simulink model "gm_minutiaeextraction_21821"  (R2018b)
settings: Solver=FixedStepDiscrete  StartTime=0.0  StopTime=10  RelTol=1e-3
undefined symbols (not defined in the file or in its folder): gray
libraries: hdlsllib x4, visionsources x1, dspmtrx3 x1
(part 2 of 7)

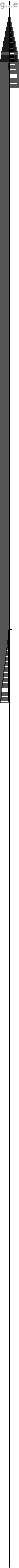
== system gm_minutiaeextraction_21821/MinutiaeFeature ==
  In1 : Inport  OutDataTypeStr=boolean  PortDimensions=[8192]  SampleTime=0.1
  MinutaeExtractTh : Subsystem
  Serializer1D1 : hdlsllib/HDL Operations/Serializer1D  Ratio=1  IdleCycles=0  validIn=off  startOut=off  validOut=off  inputDataDimensions=8192  inputSampleTime=0.1  inputSignalType=real
      settings: SourceProductName=HDL Coder  SourceProductBaseCode=HD
  concatenate{,1..63} (64 alike) : Concatenate  NumInputs=128  ConcatenateDimension=2
  concatenate64 : Concatenate  NumInputs=64  Mode=Multidimensional array  ConcatenateDimension=2
  t : Demux  Outputs=8192
  Out1 : Outport
  wires:
  In1/1 -> Serializer1D1/1
  MinutaeExtractTh/1(Out1) -> Out1/1
  concatenate64/1 -> MinutaeExtractTh/1(In1)
  Serializer1D1/1 -> t/1
  t/1 -> concatenate/1
  t/2 -> concatenate/2
  t/3 -> concatenate/3
  t/4 -> concatenate/4
  t/5 -> concatenate/5
  t/6 -> concatenate/6
  t/7 -> concatenate/7
  t/8 -> concatenate/8
  t/9 -> concatenate/9
  t/10 -> concatenate/10
  t/11 -> concatenate/11
  t/12 -> concatenate/12
  t/13 -> concatenate/13
  t/14 -> concatenate/14
  t/15 -> concatenate/15
  t/16 -> concatenate/16
  t/17 -> concatenate/17
  t/18 -> concatenate/18
  t/19 -> concatenate/19
  t/20 -> concatenate/20
  t/21 -> concatenate/21
  t/22 -> concatenate/22
  t/23 -> concatenate/23
  t/24 -> concatenate/24
  t/25 -> concatenate/25
  t/26 -> concatenate/26
  t/27 -> concatenate/27
  t/28 -> concatenate/28
  t/29 -> concatenate/29
  t/30 -> concatenate/30
  t/31 -> concatenate/31
  t/32 -> concatenate/32
  t/33 -> concatenate/33
  t/34 -> concatenate/34
  t/35 -> concatenate/35
  t/36 -> concatenate/36
  t/37 -> concatenate/37
  t/38 -> concatenate/38
  t/39 -> concatenate/39
  t/40 -> concatenate/40
  t/41 -> concatenate/41
  t/42 -> concatenate/42
  t/43 -> concatenate/43
  t/44 -> concatenate/44
  t/45 -> concatenate/45
  t/46 -> concatenate/46
  t/47 -> concatenate/47
  t/48 -> concatenate/48
  t/49 -> concatenate/49
  t/50 -> concatenate/50
  t/51 -> concatenate/51
  t/52 -> concatenate/52
  t/53 -> concatenate/53
  t/54 -> concatenate/54
  t/55 -> concatenate/55
  t/56 -> concatenate/56
  t/57 -> concatenate/57
  t/58 -> concatenate/58
  t/59 -> concatenate/59
  t/60 -> concatenate/60
  t/61 -> concatenate/61
  t/62 -> concatenate/62
  t/63 -> concatenate/63
  t/64 -> concatenate/64
  t/65 -> concatenate/65
  t/66 -> concatenate/66
  t/67 -> concatenate/67
  t/68 -> concatenate/68
  t/69 -> concatenate/69
  t/70 -> concatenate/70
  t/71 -> concatenate/71
  t/72 -> concatenate/72
  t/73 -> concatenate/73
  t/74 -> concatenate/74
  t/75 -> concatenate/75
  t/76 -> concatenate/76
  t/77 -> concatenate/77
  t/78 -> concatenate/78
  t/79 -> concatenate/79
  t/80 -> concatenate/80
  t/81 -> concatenate/81
  t/82 -> concatenate/82
  t/83 -> concatenate/83
  t/84 -> concatenate/84
  t/85 -> concatenate/85
  t/86 -> concatenate/86
  t/87 -> concatenate/87
  t/88 -> concatenate/88
  t/89 -> concatenate/89
  t/90 -> concatenate/90
  t/91 -> concatenate/91
  t/92 -> concatenate/92
  t/93 -> concatenate/93
  t/94 -> concatenate/94
  t/95 -> concatenate/95
  t/96 -> concatenate/96
  t/97 -> concatenate/97
  t/98 -> concatenate/98
  t/99 -> concatenate/99
  t/100 -> concatenate/100
  t/101 -> concatenate/101
  t/102 -> concatenate/102
  t/103 -> concatenate/103
  t/104 -> concatenate/104
  t/105 -> concatenate/105
  t/106 -> concatenate/106
  t/107 -> concatenate/107
  t/108 -> concatenate/108
  t/109 -> concatenate/109
  t/110 -> concatenate/110
  t/111 -> concatenate/111
  t/112 -> concatenate/112
  t/113 -> concatenate/113
  t/114 -> concatenate/114
  t/115 -> concatenate/115
  t/116 -> concatenate/116
  t/117 -> concatenate/117
  t/118 -> concatenate/118
  t/119 -> concatenate/119
  t/120 -> concatenate/120
  t/121 -> concatenate/121
  t/122 -> concatenate/122
  t/123 -> concatenate/123
  t/124 -> concatenate/124
  t/125 -> concatenate/125
  t/126 -> concatenate/126
  t/127 -> concatenate/127
  t/128 -> concatenate/128
  t/129 -> concatenate1/1
  t/130 -> concatenate1/2
  t/131 -> concatenate1/3
  t/132 -> concatenate1/4
  t/133 -> concatenate1/5
  t/134 -> concatenate1/6
  t/135 -> concatenate1/7
  t/136 -> concatenate1/8
  t/137 -> concatenate1/9
  t/138 -> concatenate1/10
  t/139 -> concatenate1/11
  t/140 -> concatenate1/12
  t/141 -> concatenate1/13
  t/142 -> concatenate1/14
  t/143 -> concatenate1/15
  t/144 -> concatenate1/16
  t/145 -> concatenate1/17
  t/146 -> concatenate1/18
  t/147 -> concatenate1/19
  t/148 -> concatenate1/20
  t/149 -> concatenate1/21
  t/150 -> concatenate1/22
  t/151 -> concatenate1/23
  t/152 -> concatenate1/24
  t/153 -> concatenate1/25
  t/154 -> concatenate1/26
  t/155 -> concatenate1/27
  t/156 -> concatenate1/28
  t/157 -> concatenate1/29
  t/158 -> concatenate1/30
  t/159 -> concatenate1/31
  t/160 -> concatenate1/32
  t/161 -> concatenate1/33
  t/162 -> concatenate1/34
  t/163 -> concatenate1/35
  t/164 -> concatenate1/36
  t/165 -> concatenate1/37
  t/166 -> concatenate1/38
  t/167 -> concatenate1/39
  t/168 -> concatenate1/40
  t/169 -> concatenate1/41
  t/170 -> concatenate1/42
  t/171 -> concatenate1/43
  t/172 -> concatenate1/44
  t/173 -> concatenate1/45
  t/174 -> concatenate1/46
  t/175 -> concatenate1/47
  t/176 -> concatenate1/48
  t/177 -> concatenate1/49
  t/178 -> concatenate1/50
  t/179 -> concatenate1/51
  t/180 -> concatenate1/52
  t/181 -> concatenate1/53
  t/182 -> concatenate1/54
  t/183 -> concatenate1/55
  t/184 -> concatenate1/56
  t/185 -> concatenate1/57
  t/186 -> concatenate1/58
  t/187 -> concatenate1/59
  t/188 -> concatenate1/60
  t/189 -> concatenate1/61
  t/190 -> concatenate1/62
  t/191 -> concatenate1/63
  t/192 -> concatenate1/64
  t/193 -> concatenate1/65
  t/194 -> concatenate1/66
  t/195 -> concatenate1/67
  t/196 -> concatenate1/68
  t/197 -> concatenate1/69
  t/198 -> concatenate1/70
  t/199 -> concatenate1/71
  t/200 -> concatenate1/72
  t/201 -> concatenate1/73
  t/202 -> concatenate1/74
  t/203 -> concatenate1/75
  t/204 -> concatenate1/76
  t/205 -> concatenate1/77
  t/206 -> concatenate1/78
  t/207 -> concatenate1/79
  t/208 -> concatenate1/80
  t/209 -> concatenate1/81
  t/210 -> concatenate1/82
  t/211 -> concatenate1/83
  t/212 -> concatenate1/84
  t/213 -> concatenate1/85
  t/214 -> concatenate1/86
  t/215 -> concatenate1/87
  t/216 -> concatenate1/88
  t/217 -> concatenate1/89
  t/218 -> concatenate1/90
  t/219 -> concatenate1/91
  t/220 -> concatenate1/92
  t/221 -> concatenate1/93
  t/222 -> concatenate1/94
  t/223 -> concatenate1/95
  t/224 -> concatenate1/96
  t/225 -> concatenate1/97
  t/226 -> concatenate1/98
  t/227 -> concatenate1/99
  t/228 -> concatenate1/100
  t/229 -> concatenate1/101
  t/230 -> concatenate1/102
  t/231 -> concatenate1/103
  t/232 -> concatenate1/104
  t/233 -> concatenate1/105
  t/234 -> concatenate1/106
  t/235 -> concatenate1/107
  t/236 -> concatenate1/108
  t/237 -> concatenate1/109
  t/238 -> concatenate1/110
  t/239 -> concatenate1/111
  t/240 -> concatenate1/112
  t/241 -> concatenate1/113
  t/242 -> concatenate1/114
  t/243 -> concatenate1/115
  t/244 -> concatenate1/116
  t/245 -> concatenate1/117
  t/246 -> concatenate1/118
  t/247 -> concatenate1/119
  t/248 -> concatenate1/120
  t/249 -> concatenate1/121
  t/250 -> concatenate1/122
  t/251 -> concatenate1/123
  t/252 -> concatenate1/124
  t/253 -> concatenate1/125
  t/254 -> concatenate1/126
  t/255 -> concatenate1/127
  t/256 -> concatenate1/128
  t/257 -> concatenate2/1
  t/258 -> concatenate2/2
  t/259 -> concatenate2/3
  t/260 -> concatenate2/4
  t/261 -> concatenate2/5
  t/262 -> concatenate2/6
  t/263 -> concatenate2/7
  t/264 -> concatenate2/8
  t/265 -> concatenate2/9
  t/266 -> concatenate2/10
  t/267 -> concatenate2/11
  t/268 -> concatenate2/12
  t/269 -> concatenate2/13
  t/270 -> concatenate2/14
  t/271 -> concatenate2/15
  t/272 -> concatenate2/16
  t/273 -> concatenate2/17
  t/274 -> concatenate2/18
  t/275 -> concatenate2/19
  t/276 -> concatenate2/20
  t/277 -> concatenate2/21
  t/278 -> concatenate2/22
  t/279 -> concatenate2/23
  t/280 -> concatenate2/24
  t/281 -> concatenate2/25
  t/282 -> concatenate2/26
  t/283 -> concatenate2/27
  t/284 -> concatenate2/28
  t/285 -> concatenate2/29
  t/286 -> concatenate2/30
  t/287 -> concatenate2/31
  t/288 -> concatenate2/32
  t/289 -> concatenate2/33
  t/290 -> concatenate2/34
  t/291 -> concatenate2/35
  t/292 -> concatenate2/36
  t/293 -> concatenate2/37
  t/294 -> concatenate2/38
  t/295 -> concatenate2/39
  t/296 -> concatenate2/40
  t/297 -> concatenate2/41
  t/298 -> concatenate2/42
  t/299 -> concatenate2/43
  t/300 -> concatenate2/44
  t/301 -> concatenate2/45
  t/302 -> concatenate2/46
  t/303 -> concatenate2/47
  t/304 -> concatenate2/48
  t/305 -> concatenate2/49
  t/306 -> concatenate2/50
  t/307 -> concatenate2/51
  t/308 -> concatenate2/52
  t/309 -> concatenate2/53
  t/310 -> concatenate2/54
  t/311 -> concatenate2/55
  t/312 -> concatenate2/56
  t/313 -> concatenate2/57
  t/314 -> concatenate2/58
  t/315 -> concatenate2/59
  t/316 -> concatenate2/60
  t/317 -> concatenate2/61
  t/318 -> concatenate2/62
  t/319 -> concatenate2/63
  t/320 -> concatenate2/64
  t/321 -> concatenate2/65
  t/322 -> concatenate2/66
  t/323 -> concatenate2/67
  t/324 -> concatenate2/68
  t/325 -> concatenate2/69
  t/326 -> concatenate2/70
  t/327 -> concatenate2/71
  t/328 -> concatenate2/72
  t/329 -> concatenate2/73
  t/330 -> concatenate2/74
  t/331 -> concatenate2/75
  t/332 -> concatenate2/76
  t/333 -> concatenate2/77
  t/334 -> concatenate2/78
  t/335 -> concatenate2/79
  t/336 -> concatenate2/80
  t/337 -> concatenate2/81
  t/338 -> concatenate2/82
  t/339 -> concatenate2/83
  t/340 -> concatenate2/84
  t/341 -> concatenate2/85
  t/342 -> concatenate2/86
  t/343 -> concatenate2/87
  t/344 -> concatenate2/88
  t/345 -> concatenate2/89
  t/346 -> concatenate2/90
  t/347 -> concatenate2/91
  t/348 -> concatenate2/92
  t/349 -> concatenate2/93
  t/350 -> concatenate2/94
  t/351 -> concatenate2/95
  t/352 -> concatenate2/96
  t/353 -> concatenate2/97
  t/354 -> concatenate2/98
  t/355 -> concatenate2/99
  t/356 -> concatenate2/100
  t/357 -> concatenate2/101
  t/358 -> concatenate2/102
  t/359 -> concatenate2/103
  t/360 -> concatenate2/104
  t/361 -> concatenate2/105
  t/362 -> concatenate2/106
  t/363 -> concatenate2/107
  t/364 -> concatenate2/108
  t/365 -> concatenate2/109
  t/366 -> concatenate2/110
  t/367 -> concatenate2/111
  t/368 -> concatenate2/112
  t/369 -> concatenate2/113
  t/370 -> concatenate2/114
  t/371 -> concatenate2/115
  t/372 -> concatenate2/116
  t/373 -> concatenate2/117
  t/374 -> concatenate2/118
  t/375 -> concatenate2/119
  t/376 -> concatenate2/120
  t/377 -> concatenate2/121
  t/378 -> concatenate2/122
  t/379 -> concatenate2/123
  t/380 -> concatenate2/124
  t/381 -> concatenate2/125
  t/382 -> concatenate2/126
  t/383 -> concatenate2/127
  t/384 -> concatenate2/128
  t/385 -> concatenate3/1
  t/386 -> concatenate3/2
  t/387 -> concatenate3/3
  t/388 -> concatenate3/4
  t/389 -> concatenate3/5
  t/390 -> concatenate3/6
  t/391 -> concatenate3/7
  t/392 -> concatenate3/8
  t/393 -> concatenate3/9
  t/394 -> concatenate3/10
  t/395 -> concatenate3/11
  t/396 -> concatenate3/12
  t/397 -> concatenate3/13
  t/398 -> concatenate3/14
  t/399 -> concatenate3/15
  t/400 -> concatenate3/16
  t/401 -> concatenate3/17
  t/402 -> concatenate3/18
  t/403 -> concatenate3/19
  t/404 -> concatenate3/20
  t/405 -> concatenate3/21
  t/406 -> concatenate3/22
  t/407 -> concatenate3/23
  t/408 -> concatenate3/24
  t/409 -> concatenate3/25
  t/410 -> concatenate3/26
  t/411 -> concatenate3/27
  t/412 -> concatenate3/28
  t/413 -> concatenate3/29
  t/414 -> concatenate3/30
  t/415 -> concatenate3/31
  t/416 -> concatenate3/32
  t/417 -> concatenate3/33
  t/418 -> concatenate3/34
  t/419 -> concatenate3/35
  t/420 -> concatenate3/36
  t/421 -> concatenate3/37
  t/422 -> concatenate3/38
  t/423 -> concatenate3/39
  t/424 -> concatenate3/40
  t/425 -> concatenate3/41
  t/426 -> concatenate3/42
  t/427 -> concatenate3/43
  t/428 -> concatenate3/44
  t/429 -> concatenate3/45
  t/430 -> concatenate3/46
  t/431 -> concatenate3/47
  t/432 -> concatenate3/48
  t/433 -> concatenate3/49
  t/434 -> concatenate3/50
  t/435 -> concatenate3/51
  t/436 -> concatenate3/52
  t/437 -> concatenate3/53
  t/438 -> concatenate3/54
  t/439 -> concatenate3/55
  t/440 -> concatenate3/56
  t/441 -> concatenate3/57
  t/442 -> concatenate3/58
  t/443 -> concatenate3/59
  t/444 -> concatenate3/60
  t/445 -> concatenate3/61
  t/446 -> concatenate3/62
  t/447 -> concatenate3/63
  t/448 -> concatenate3/64
  t/449 -> concatenate3/65
  t/450 -> concatenate3/66
  t/451 -> concatenate3/67
  t/452 -> concatenate3/68
  t/453 -> concatenate3/69
  t/454 -> concatenate3/70
  t/455 -> concatenate3/71
  t/456 -> concatenate3/72
  t/457 -> concatenate3/73
  t/458 -> concatenate3/74
  t/459 -> concatenate3/75
  t/460 -> concatenate3/76
  t/461 -> concatenate3/77
  t/462 -> concatenate3/78
  t/463 -> concatenate3/79
  t/464 -> concatenate3/80
  t/465 -> concatenate3/81
  t/466 -> concatenate3/82
  t/467 -> concatenate3/83
  t/468 -> concatenate3/84
  t/469 -> concatenate3/85
  t/470 -> concatenate3/86
  t/471 -> concatenate3/87
  t/472 -> concatenate3/88
  t/473 -> concatenate3/89
  t/474 -> concatenate3/90
  t/475 -> concatenate3/91
  t/476 -> concatenate3/92
  t/477 -> concatenate3/93
  t/478 -> concatenate3/94
  t/479 -> concatenate3/95
  t/480 -> concatenate3/96
  t/481 -> concatenate3/97
  t/482 -> concatenate3/98
  t/483 -> concatenate3/99
  t/484 -> concatenate3/100
  t/485 -> concatenate3/101
  t/486 -> concatenate3/102
  t/487 -> concatenate3/103
  t/488 -> concatenate3/104
  t/489 -> concatenate3/105
  t/490 -> concatenate3/106
  t/491 -> concatenate3/107
  t/492 -> concatenate3/108
  t/493 -> concatenate3/109
  t/494 -> concatenate3/110
  t/495 -> concatenate3/111
  t/496 -> concatenate3/112
  t/497 -> concatenate3/113
  t/498 -> concatenate3/114
  t/499 -> concatenate3/115
  t/500 -> concatenate3/116
  t/501 -> concatenate3/117
  t/502 -> concatenate3/118
  t/503 -> concatenate3/119
  t/504 -> concatenate3/120
  t/505 -> concatenate3/121
  t/506 -> concatenate3/122
  t/507 -> concatenate3/123
  t/508 -> concatenate3/124
  t/509 -> concatenate3/125
  t/510 -> concatenate3/126
  t/511 -> concatenate3/127
  t/512 -> concatenate3/128
  t/513 -> concatenate4/1
  t/514 -> concatenate4/2
  t/515 -> concatenate4/3
  t/516 -> concatenate4/4
  t/517 -> concatenate4/5
  t/518 -> concatenate4/6
  t/519 -> concatenate4/7
  t/520 -> concatenate4/8
  t/521 -> concatenate4/9
  t/522 -> concatenate4/10
  t/523 -> concatenate4/11
  t/524 -> concatenate4/12
  t/525 -> concatenate4/13
  t/526 -> concatenate4/14
  t/527 -> concatenate4/15
  t/528 -> concatenate4/16
  t/529 -> concatenate4/17
  t/530 -> concatenate4/18
  t/531 -> concatenate4/19
  t/532 -> concatenate4/20
  t/533 -> concatenate4/21
  t/534 -> concatenate4/22
  t/535 -> concatenate4/23
  t/536 -> concatenate4/24
  t/537 -> concatenate4/25
  t/538 -> concatenate4/26
  t/539 -> concatenate4/27
  t/540 -> concatenate4/28
  t/541 -> concatenate4/29
  t/542 -> concatenate4/30
  t/543 -> concatenate4/31
  t/544 -> concatenate4/32
  t/545 -> concatenate4/33
  t/546 -> concatenate4/34
  t/547 -> concatenate4/35
  t/548 -> concatenate4/36
  t/549 -> concatenate4/37
  t/550 -> concatenate4/38
  t/551 -> concatenate4/39
  t/552 -> concatenate4/40
  t/553 -> concatenate4/41
  t/554 -> concatenate4/42
  t/555 -> concatenate4/43
  t/556 -> concatenate4/44
  t/557 -> concatenate4/45
  t/558 -> concatenate4/46
  t/559 -> concatenate4/47
  t/560 -> concatenate4/48
  t/561 -> concatenate4/49
  t/562 -> concatenate4/50
  t/563 -> concatenate4/51
  t/564 -> concatenate4/52
  t/565 -> concatenate4/53
  t/566 -> concatenate4/54
  t/567 -> concatenate4/55
  t/568 -> concatenate4/56
  t/569 -> concatenate4/57
  t/570 -> concatenate4/58
  t/571 -> concatenate4/59
  t/572 -> concatenate4/60
  t/573 -> concatenate4/61
  t/574 -> concatenate4/62
  t/575 -> concatenate4/63
  t/576 -> concatenate4/64
  t/577 -> concatenate4/65
  t/578 -> concatenate4/66
  t/579 -> concatenate4/67
  t/580 -> concatenate4/68
  t/581 -> concatenate4/69
  t/582 -> concatenate4/70
  t/583 -> concatenate4/71
  t/584 -> concatenate4/72
  t/585 -> concatenate4/73
  t/586 -> concatenate4/74
  t/587 -> concatenate4/75
  t/588 -> concatenate4/76
  t/589 -> concatenate4/77
  t/590 -> concatenate4/78
  t/591 -> concatenate4/79
  t/592 -> concatenate4/80
  t/593 -> concatenate4/81
  t/594 -> concatenate4/82
  t/595 -> concatenate4/83
  t/596 -> concatenate4/84
  t/597 -> concatenate4/85
  t/598 -> concatenate4/86
  t/599 -> concatenate4/87
  t/600 -> concatenate4/88
  t/601 -> concatenate4/89
  t/602 -> concatenate4/90
  t/603 -> concatenate4/91
  t/604 -> concatenate4/92
  t/605 -> concatenate4/93
  t/606 -> concatenate4/94
  t/607 -> concatenate4/95
  t/608 -> concatenate4/96
  t/609 -> concatenate4/97
  t/610 -> concatenate4/98
  t/611 -> concatenate4/99
  t/612 -> concatenate4/100
  t/613 -> concatenate4/101
  t/614 -> concatenate4/102
  t/615 -> concatenate4/103
  t/616 -> concatenate4/104
  t/617 -> concatenate4/105
  t/618 -> concatenate4/106
  t/619 -> concatenate4/107
  t/620 -> concatenate4/108
  t/621 -> concatenate4/109
  t/622 -> concatenate4/110
  t/623 -> concatenate4/111
  t/624 -> concatenate4/112
  t/625 -> concatenate4/113
  t/626 -> concatenate4/114
  t/627 -> concatenate4/115
  t/628 -> concatenate4/116
  t/629 -> concatenate4/117
  t/630 -> concatenate4/118
  t/631 -> concatenate4/119
  t/632 -> concatenate4/120
  t/633 -> concatenate4/121
  t/634 -> concatenate4/122
  t/635 -> concatenate4/123
  t/636 -> concatenate4/124
  t/637 -> concatenate4/125
  t/638 -> concatenate4/126
  t/639 -> concatenate4/127
  t/640 -> concatenate4/128
  t/641 -> concatenate5/1
  t/642 -> concatenate5/2
  t/643 -> concatenate5/3
  t/644 -> concatenate5/4
  t/645 -> concatenate5/5
  t/646 -> concatenate5/6
  t/647 -> concatenate5/7
  t/648 -> concatenate5/8
  t/649 -> concatenate5/9
  t/650 -> concatenate5/10
  t/651 -> concatenate5/11
  t/652 -> concatenate5/12
  t/653 -> concatenate5/13
  t/654 -> concatenate5/14
  t/655 -> concatenate5/15
  t/656 -> concatenate5/16
  t/657 -> concatenate5/17
  t/658 -> concatenate5/18
  t/659 -> concatenate5/19
  t/660 -> concatenate5/20
  t/661 -> concatenate5/21
  t/662 -> concatenate5/22
  t/663 -> concatenate5/23
  t/664 -> concatenate5/24
  t/665 -> concatenate5/25
  t/666 -> concatenate5/26
  t/667 -> concatenate5/27
  t/668 -> concatenate5/28
  t/669 -> concatenate5/29
  t/670 -> concatenate5/30
  t/671 -> concatenate5/31
  t/672 -> concatenate5/32
  t/673 -> concatenate5/33
  t/674 -> concatenate5/34
  t/675 -> concatenate5/35
  t/676 -> concatenate5/36
  t/677 -> concatenate5/37
  t/678 -> concatenate5/38
  t/679 -> concatenate5/39
  t/680 -> concatenate5/40
  t/681 -> concatenate5/41
  t/682 -> concatenate5/42
  t/683 -> concatenate5/43
  t/684 -> concatenate5/44
  t/685 -> concatenate5/45
  t/686 -> concatenate5/46
  t/687 -> concatenate5/47
  t/688 -> concatenate5/48
  t/689 -> concatenate5/49
  t/690 -> concatenate5/50
  t/691 -> concatenate5/51
  t/692 -> concatenate5/52
  t/693 -> concatenate5/53
  t/694 -> concatenate5/54
  t/695 -> concatenate5/55
  t/696 -> concatenate5/56
  t/697 -> concatenate5/57
  t/698 -> concatenate5/58
  t/699 -> concatenate5/59
  t/700 -> concatenate5/60
  t/701 -> concatenate5/61
  t/702 -> concatenate5/62
  t/703 -> concatenate5/63
  t/704 -> concatenate5/64
  t/705 -> concatenate5/65
  t/706 -> concatenate5/66
  t/707 -> concatenate5/67
  t/708 -> concatenate5/68
  t/709 -> concatenate5/69
  t/710 -> concatenate5/70
  t/711 -> concatenate5/71
  t/712 -> concatenate5/72
  t/713 -> concatenate5/73
  t/714 -> concatenate5/74
  t/715 -> concatenate5/75
  t/716 -> concatenate5/76
  t/717 -> concatenate5/77
  t/718 -> concatenate5/78
  t/719 -> concatenate5/79
  t/720 -> concatenate5/80
  t/721 -> concatenate5/81
  t/722 -> concatenate5/82
  t/723 -> concatenate5/83
  t/724 -> concatenate5/84
  t/725 -> concatenate5/85
  t/726 -> concatenate5/86
  t/727 -> concatenate5/87
  t/728 -> concatenate5/88
  t/729 -> concatenate5/89
  t/730 -> concatenate5/90
  t/731 -> concatenate5/91
  t/732 -> concatenate5/92
  t/733 -> concatenate5/93
  t/734 -> concatenate5/94
  t/735 -> concatenate5/95
  t/736 -> concatenate5/96
  t/737 -> concatenate5/97
  t/738 -> concatenate5/98
  t/739 -> concatenate5/99
  t/740 -> concatenate5/100
  t/741 -> concatenate5/101
  t/742 -> concatenate5/102
  t/743 -> concatenate5/103
  t/744 -> concatenate5/104
  t/745 -> concatenate5/105
  t/746 -> concatenate5/106
  t/747 -> concatenate5/107
  t/748 -> concatenate5/108
  t/749 -> concatenate5/109
  t/750 -> concatenate5/110
  t/751 -> concatenate5/111
  t/752 -> concatenate5/112
  t/753 -> concatenate5/113
  t/754 -> concatenate5/114
  t/755 -> concatenate5/115
  t/756 -> concatenate5/116
  t/757 -> concatenate5/117
  t/758 -> concatenate5/118
  t/759 -> concatenate5/119
  t/760 -> concatenate5/120
  t/761 -> concatenate5/121
  t/762 -> concatenate5/122
  t/763 -> concatenate5/123
  t/764 -> concatenate5/124
  t/765 -> concatenate5/125
  t/766 -> concatenate5/126
  t/767 -> concatenate5/127
  t/768 -> concatenate5/128
  t/769 -> concatenate6/1
  t/770 -> concatenate6/2
  t/771 -> concatenate6/3
  t/772 -> concatenate6/4
  t/773 -> concatenate6/5
  t/774 -> concatenate6/6
  t/775 -> concatenate6/7
  t/776 -> concatenate6/8
  t/777 -> concatenate6/9
  t/778 -> concatenate6/10
  t/779 -> concatenate6/11
  t/780 -> concatenate6/12
  t/781 -> concatenate6/13
  t/782 -> concatenate6/14
  t/783 -> concatenate6/15
  t/784 -> concatenate6/16
  t/785 -> concatenate6/17
  t/786 -> concatenate6/18
  t/787 -> concatenate6/19
  t/788 -> concatenate6/20
  t/789 -> concatenate6/21
  t/790 -> concatenate6/22
  t/791 -> concatenate6/23
  t/792 -> concatenate6/24
  t/793 -> concatenate6/25
  t/794 -> concatenate6/26
  t/795 -> concatenate6/27
  t/796 -> concatenate6/28
  t/797 -> concatenate6/29
  t/798 -> concatenate6/30
  t/799 -> concatenate6/31
  t/800 -> concatenate6/32
  t/801 -> concatenate6/33
  t/802 -> concatenate6/34
  t/803 -> concatenate6/35
  t/804 -> concatenate6/36
  t/805 -> concatenate6/37
  t/806 -> concatenate6/38
  t/807 -> concatenate6/39
  t/808 -> concatenate6/40
  t/809 -> concatenate6/41
  t/810 -> concatenate6/42
  t/811 -> concatenate6/43
  t/812 -> concatenate6/44
  t/813 -> concatenate6/45
  t/814 -> concatenate6/46
  t/815 -> concatenate6/47
  t/816 -> concatenate6/48
  t/817 -> concatenate6/49
  t/818 -> concatenate6/50
  t/819 -> concatenate6/51
  t/820 -> concatenate6/52
  t/821 -> concatenate6/53
  t/822 -> concatenate6/54
  t/823 -> concatenate6/55
  t/824 -> concatenate6/56
  t/825 -> concatenate6/57
  t/826 -> concatenate6/58
  t/827 -> concatenate6/59
  t/828 -> concatenate6/60
  t/829 -> concatenate6/61
  t/830 -> concatenate6/62
  t/831 -> concatenate6/63
  t/832 -> concatenate6/64
  t/833 -> concatenate6/65
  t/834 -> concatenate6/66
  t/835 -> concatenate6/67
  t/836 -> concatenate6/68
  t/837 -> concatenate6/69
  t/838 -> concatenate6/70
  t/839 -> concatenate6/71
  t/840 -> concatenate6/72
  t/841 -> concatenate6/73
  t/842 -> concatenate6/74
  t/843 -> concatenate6/75
  t/844 -> concatenate6/76
  t/845 -> concatenate6/77
  t/846 -> concatenate6/78
  t/847 -> concatenate6/79
  t/848 -> concatenate6/80
  t/849 -> concatenate6/81
  t/850 -> concatenate6/82
  t/851 -> concatenate6/83
  t/852 -> concatenate6/84
  t/853 -> concatenate6/85
  t/854 -> concatenate6/86
  t/855 -> concatenate6/87
  t/856 -> concatenate6/88
  t/857 -> concatenate6/89
  t/858 -> concatenate6/90
  t/859 -> concatenate6/91
  t/860 -> concatenate6/92
  t/861 -> concatenate6/93
  t/862 -> concatenate6/94
  t/863 -> concatenate6/95
  t/864 -> concatenate6/96
  t/865 -> concatenate6/97
  t/866 -> concatenate6/98
  t/867 -> concatenate6/99
  t/868 -> concatenate6/100
  t/869 -> concatenate6/101
  t/870 -> concatenate6/102
  t/871 -> concatenate6/103
  t/872 -> concatenate6/104
  t/873 -> concatenate6/105
  t/874 -> concatenate6/106
  t/875 -> concatenate6/107
  t/876 -> concatenate6/108
  t/877 -> concatenate6/109
  t/878 -> concatenate6/110
  t/879 -> concatenate6/111
  t/880 -> concatenate6/112
  t/881 -> concatenate6/113
  t/882 -> concatenate6/114
  t/883 -> concatenate6/115
  t/884 -> concatenate6/116
  t/885 -> concatenate6/117
  t/886 -> concatenate6/118
  t/887 -> concatenate6/119
  t/888 -> concatenate6/120
  t/889 -> concatenate6/121
  t/890 -> concatenate6/122
  t/891 -> concatenate6/123
  t/892 -> concatenate6/124
  t/893 -> concatenate6/125
  t/894 -> concatenate6/126
  t/895 -> concatenate6/127
  t/896 -> concatenate6/128
  t/897 -> concatenate7/1
  t/898 -> concatenate7/2
  t/899 -> concatenate7/3
  t/900 -> concatenate7/4
  t/901 -> concatenate7/5
  t/902 -> concatenate7/6
  t/903 -> concatenate7/7
  t/904 -> concatenate7/8
  t/905 -> concatenate7/9
  t/906 -> concatenate7/10
  t/907 -> concatenate7/11
  t/908 -> concatenate7/12
  t/909 -> concatenate7/13
  t/910 -> concatenate7/14
  t/911 -> concatenate7/15
  t/912 -> concatenate7/16
  t/913 -> concatenate7/17
  t/914 -> concatenate7/18
  t/915 -> concatenate7/19
  t/916 -> concatenate7/20
  t/917 -> concatenate7/21
  t/918 -> concatenate7/22
  t/919 -> concatenate7/23
  t/920 -> concatenate7/24
  t/921 -> concatenate7/25
  t/922 -> concatenate7/26
  t/923 -> concatenate7/27
  t/924 -> concatenate7/28
  t/925 -> concatenate7/29
  t/926 -> concatenate7/30
  t/927 -> concatenate7/31
  t/928 -> concatenate7/32
  t/929 -> concatenate7/33
  t/930 -> concatenate7/34
  t/931 -> concatenate7/35
  t/932 -> concatenate7/36
  t/933 -> concatenate7/37
  t/934 -> concatenate7/38
  t/935 -> concatenate7/39
  t/936 -> concatenate7/40
  t/937 -> concatenate7/41
  t/938 -> concatenate7/42
  t/939 -> concatenate7/43
  t/940 -> concatenate7/44
  t/941 -> concatenate7/45
  t/942 -> concatenate7/46
  t/943 -> concatenate7/47
  t/944 -> concatenate7/48
  t/945 -> concatenate7/49
  t/946 -> concatenate7/50
  t/947 -> concatenate7/51
  t/948 -> concatenate7/52
  t/949 -> concatenate7/53
  t/950 -> concatenate7/54
  t/951 -> concatenate7/55
  t/952 -> concatenate7/56
  t/953 -> concatenate7/57
  t/954 -> concatenate7/58
  t/955 -> concatenate7/59
  t/956 -> concatenate7/60
  t/957 -> concatenate7/61
  t/958 -> concatenate7/62
  t/959 -> concatenate7/63
  t/960 -> concatenate7/64
  t/961 -> concatenate7/65
  t/962 -> concatenate7/66
  t/963 -> concatenate7/67
  t/964 -> concatenate7/68
  t/965 -> concatenate7/69
  t/966 -> concatenate7/70
  t/967 -> concatenate7/71
  t/968 -> concatenate7/72
  t/969 -> concatenate7/73
  t/970 -> concatenate7/74
  t/971 -> concatenate7/75
  t/972 -> concatenate7/76
  t/973 -> concatenate7/77
  t/974 -> concatenate7/78
  t/975 -> concatenate7/79
  t/976 -> concatenate7/80
  t/977 -> concatenate7/81
  t/978 -> concatenate7/82
  t/979 -> concatenate7/83
  t/980 -> concatenate7/84
  t/981 -> concatenate7/85
  t/982 -> concatenate7/86
  t/983 -> concatenate7/87
  t/984 -> concatenate7/88
  t/985 -> concatenate7/89
  t/986 -> concatenate7/90
  t/987 -> concatenate7/91
  t/988 -> concatenate7/92
  t/989 -> concatenate7/93
  t/990 -> concatenate7/94
  t/991 -> concatenate7/95
  t/992 -> concatenate7/96
  t/993 -> concatenate7/97
  t/994 -> concatenate7/98
  t/995 -> concatenate7/99
  t/996 -> concatenate7/100
  t/997 -> concatenate7/101
  t/998 -> concatenate7/102
  t/999 -> concatenate7/103
  t/1000 -> concatenate7/104
  t/1001 -> concatenate7/105
  t/1002 -> concatenate7/106
  t/1003 -> concatenate7/107
  t/1004 -> concatenate7/108
  t/1005 -> concatenate7/109
  t/1006 -> concatenate7/110
  t/1007 -> concatenate7/111
  t/1008 -> concatenate7/112
  t/1009 -> concatenate7/113
  t/1010 -> concatenate7/114
  t/1011 -> concatenate7/115
  t/1012 -> concatenate7/116
  t/1013 -> concatenate7/117
  t/1014 -> concatenate7/118
  t/1015 -> concatenate7/119
  t/1016 -> concatenate7/120
  t/1017 -> concatenate7/121
  t/1018 -> concatenate7/122
  t/1019 -> concatenate7/123
  t/1020 -> concatenate7/124
  t/1021 -> concatenate7/125
  t/1022 -> concatenate7/126
  t/1023 -> concatenate7/127
  t/1024 -> concatenate7/128
  t/1025 -> concatenate8/1
  t/1026 -> concatenate8/2
  t/1027 -> concatenate8/3
  t/1028 -> concatenate8/4
  t/1029 -> concatenate8/5
  t/1030 -> concatenate8/6
  t/1031 -> concatenate8/7
  t/1032 -> concatenate8/8
  t/1033 -> concatenate8/9
  t/1034 -> concatenate8/10
  t/1035 -> concatenate8/11
  t/1036 -> concatenate8/12
  t/1037 -> concatenate8/13
  t/1038 -> concatenate8/14
  t/1039 -> concatenate8/15
  t/1040 -> concatenate8/16
  t/1041 -> concatenate8/17
  t/1042 -> concatenate8/18
  t/1043 -> concatenate8/19
  t/1044 -> concatenate8/20
  t/1045 -> concatenate8/21
  t/1046 -> concatenate8/22
  t/1047 -> concatenate8/23
  t/1048 -> concatenate8/24
  t/1049 -> concatenate8/25
  t/1050 -> concatenate8/26
  t/1051 -> concatenate8/27
  t/1052 -> concatenate8/28
  t/1053 -> concatenate8/29
  t/1054 -> concatenate8/30
  t/1055 -> concatenate8/31
  t/1056 -> concatenate8/32
  t/1057 -> concatenate8/33
  t/1058 -> concatenate8/34
  t/1059 -> concatenate8/35
  t/1060 -> concatenate8/36
  t/1061 -> concatenate8/37
  t/1062 -> concatenate8/38
  t/1063 -> concatenate8/39
  t/1064 -> concatenate8/40
  t/1065 -> concatenate8/41
  t/1066 -> concatenate8/42
  t/1067 -> concatenate8/43
  t/1068 -> concatenate8/44
  t/1069 -> concatenate8/45
  t/1070 -> concatenate8/46
  t/1071 -> concatenate8/47
  t/1072 -> concatenate8/48
  t/1073 -> concatenate8/49
  t/1074 -> concatenate8/50
  t/1075 -> concatenate8/51
  t/1076 -> concatenate8/52
  t/1077 -> concatenate8/53
  t/1078 -> concatenate8/54
  t/1079 -> concatenate8/55
  t/1080 -> concatenate8/56
  t/1081 -> concatenate8/57
  t/1082 -> concatenate8/58
  t/1083 -> concatenate8/59
  t/1084 -> concatenate8/60
  t/1085 -> concatenate8/61
  t/1086 -> concatenate8/62
  t/1087 -> concatenate8/63
  t/1088 -> concatenate8/64
  t/1089 -> concatenate8/65
  t/1090 -> concatenate8/66
  t/1091 -> concatenate8/67
  t/1092 -> concatenate8/68
  t/1093 -> concatenate8/69
  t/1094 -> concatenate8/70
  t/1095 -> concatenate8/71
  t/1096 -> concatenate8/72
  t/1097 -> concatenate8/73
  t/1098 -> concatenate8/74
  t/1099 -> concatenate8/75
  t/1100 -> concatenate8/76
  t/1101 -> concatenate8/77
  t/1102 -> concatenate8/78
  t/1103 -> concatenate8/79
  t/1104 -> concatenate8/80
  t/1105 -> concatenate8/81
  t/1106 -> concatenate8/82
  t/1107 -> concatenate8/83
  t/1108 -> concatenate8/84
  t/1109 -> concatenate8/85
  t/1110 -> concatenate8/86
  t/1111 -> concatenate8/87
  t/1112 -> concatenate8/88
  t/1113 -> concatenate8/89
  t/1114 -> concatenate8/90
  t/1115 -> concatenate8/91
  t/1116 -> concatenate8/92
  t/1117 -> concatenate8/93
  t/1118 -> concatenate8/94
  t/1119 -> concatenate8/95
  t/1120 -> concatenate8/96
  t/1121 -> concatenate8/97
  t/1122 -> concatenate8/98
  t/1123 -> concatenate8/99
  t/1124 -> concatenate8/100
  t/1125 -> concatenate8/101
  t/1126 -> concatenate8/102
  t/1127 -> concatenate8/103
  t/1128 -> concatenate8/104
  t/1129 -> concatenate8/105
  t/1130 -> concatenate8/106
  t/1131 -> concatenate8/107
  t/1132 -> concatenate8/108
  t/1133 -> concatenate8/109
  t/1134 -> concatenate8/110
  t/1135 -> concatenate8/111
  t/1136 -> concatenate8/112
  t/1137 -> concatenate8/113
  t/1138 -> concatenate8/114
  t/1139 -> concatenate8/115
  t/1140 -> concatenate8/116
  t/1141 -> concatenate8/117
  t/1142 -> concatenate8/118
  t/1143 -> concatenate8/119
  t/1144 -> concatenate8/120
  t/1145 -> concatenate8/121
  t/1146 -> concatenate8/122
  t/1147 -> concatenate8/123
  t/1148 -> concatenate8/124
  t/1149 -> concatenate8/125
  t/1150 -> concatenate8/126
  t/1151 -> concatenate8/127
  t/1152 -> concatenate8/128
  t/1153 -> concatenate9/1
  t/1154 -> concatenate9/2
  t/1155 -> concatenate9/3
  t/1156 -> concatenate9/4
  t/1157 -> concatenate9/5
  t/1158 -> concatenate9/6
  t/1159 -> concatenate9/7
  t/1160 -> concatenate9/8
  t/1161 -> concatenate9/9
  t/1162 -> concatenate9/10
  t/1163 -> concatenate9/11
  t/1164 -> concatenate9/12
  t/1165 -> concatenate9/13
  t/1166 -> concatenate9/14
  t/1167 -> concatenate9/15
  t/1168 -> concatenate9/16
  t/1169 -> concatenate9/17
  t/1170 -> concatenate9/18
  t/1171 -> concatenate9/19
  t/1172 -> concatenate9/20
  t/1173 -> concatenate9/21
  t/1174 -> concatenate9/22
  t/1175 -> concatenate9/23
  t/1176 -> concatenate9/24
  t/1177 -> concatenate9/25
  t/1178 -> concatenate9/26
  t/1179 -> concatenate9/27
  t/1180 -> concatenate9/28
  t/1181 -> concatenate9/29
  t/1182 -> concatenate9/30
  t/1183 -> concatenate9/31
  t/1184 -> concatenate9/32
  t/1185 -> concatenate9/33
  t/1186 -> concatenate9/34
  t/1187 -> concatenate9/35
  t/1188 -> concatenate9/36
  t/1189 -> concatenate9/37
  t/1190 -> concatenate9/38
  t/1191 -> concatenate9/39
  t/1192 -> concatenate9/40
  t/1193 -> concatenate9/41
  t/1194 -> concatenate9/42
  t/1195 -> concatenate9/43
  t/1196 -> concatenate9/44
  t/1197 -> concatenate9/45
  t/1198 -> concatenate9/46
  t/1199 -> concatenate9/47
  t/1200 -> concatenate9/48
  t/1201 -> concatenate9/49
  t/1202 -> concatenate9/50
  t/1203 -> concatenate9/51
  t/1204 -> concatenate9/52
  t/1205 -> concatenate9/53
  t/1206 -> concatenate9/54
  t/1207 -> concatenate9/55
  t/1208 -> concatenate9/56
  t/1209 -> concatenate9/57
  t/1210 -> concatenate9/58
  t/1211 -> concatenate9/59
  t/1212 -> concatenate9/60
  t/1213 -> concatenate9/61
  t/1214 -> concatenate9/62
  t/1215 -> concatenate9/63
  t/1216 -> concatenate9/64
  t/1217 -> concatenate9/65
  t/1218 -> concatenate9/66
  t/1219 -> concatenate9/67
  t/1220 -> concatenate9/68
  t/1221 -> concatenate9/69
  t/1222 -> concatenate9/70
  t/1223 -> concatenate9/71
  t/1224 -> concatenate9/72
  t/1225 -> concatenate9/73
  t/1226 -> concatenate9/74
  t/1227 -> concatenate9/75
  t/1228 -> concatenate9/76
  t/1229 -> concatenate9/77
  t/1230 -> concatenate9/78
  t/1231 -> concatenate9/79
  t/1232 -> concatenate9/80
  t/1233 -> concatenate9/81
  t/1234 -> concatenate9/82
  t/1235 -> concatenate9/83
  t/1236 -> concatenate9/84
  t/1237 -> concatenate9/85
  t/1238 -> concatenate9/86
  t/1239 -> concatenate9/87
  t/1240 -> concatenate9/88
  t/1241 -> concatenate9/89
  t/1242 -> concatenate9/90
  t/1243 -> concatenate9/91
  t/1244 -> concatenate9/92
  t/1245 -> concatenate9/93
  t/1246 -> concatenate9/94
  t/1247 -> concatenate9/95
  t/1248 -> concatenate9/96
  t/1249 -> concatenate9/97
  t/1250 -> concatenate9/98
  t/1251 -> concatenate9/99
  t/1252 -> concatenate9/100
  t/1253 -> concatenate9/101
  t/1254 -> concatenate9/102
  t/1255 -> concatenate9/103
  t/1256 -> concatenate9/104
  t/1257 -> concatenate9/105
  t/1258 -> concatenate9/106
  t/1259 -> concatenate9/107
  t/1260 -> concatenate9/108
  t/1261 -> concatenate9/109
  t/1262 -> concatenate9/110
  t/1263 -> concatenate9/111
  t/1264 -> concatenate9/112
  t/1265 -> concatenate9/113
  t/1266 -> concatenate9/114
  t/1267 -> concatenate9/115
  t/1268 -> concatenate9/116
  t/1269 -> concatenate9/117
  t/1270 -> concatenate9/118
  t/1271 -> concatenate9/119
  t/1272 -> concatenate9/120
  t/1273 -> concatenate9/121
  t/1274 -> concatenate9/122
  t/1275 -> concatenate9/123
  t/1276 -> concatenate9/124
  t/1277 -> concatenate9/125
  t/1278 -> concatenate9/126
  t/1279 -> concatenate9/127
  t/1280 -> concatenate9/128
  t/1281 -> concatenate10/1
  t/1282 -> concatenate10/2
  t/1283 -> concatenate10/3
  t/1284 -> concatenate10/4
  t/1285 -> concatenate10/5
  t/1286 -> concatenate10/6
  t/1287 -> concatenate10/7
  t/1288 -> concatenate10/8
  t/1289 -> concatenate10/9
  t/1290 -> concatenate10/10
  t/1291 -> concatenate10/11
  t/1292 -> concatenate10/12
  t/1293 -> concatenate10/13
  t/1294 -> concatenate10/14
  t/1295 -> concatenate10/15
  t/1296 -> concatenate10/16
  t/1297 -> concatenate10/17
  t/1298 -> concatenate10/18
  t/1299 -> concatenate10/19
  t/1300 -> concatenate10/20
  t/1301 -> concatenate10/21
  t/1302 -> concatenate10/22
  t/1303 -> concatenate10/23
  t/1304 -> concatenate10/24
  t/1305 -> concatenate10/25
  t/1306 -> concatenate10/26
  t/1307 -> concatenate10/27
  t/1308 -> concatenate10/28
  t/1309 -> concatenate10/29
  t/1310 -> concatenate10/30
  t/1311 -> concatenate10/31
  t/1312 -> concatenate10/32
  t/1313 -> concatenate10/33
  t/1314 -> concatenate10/34
  t/1315 -> concatenate10/35
  t/1316 -> concatenate10/36
  t/1317 -> concatenate10/37
  t/1318 -> concatenate10/38
  t/1319 -> concatenate10/39
  t/1320 -> concatenate10/40
  t/1321 -> concatenate10/41
  t/1322 -> concatenate10/42
  t/1323 -> concatenate10/43
  t/1324 -> concatenate10/44
  t/1325 -> concatenate10/45
  t/1326 -> concatenate10/46
  t/1327 -> concatenate10/47
  t/1328 -> concatenate10/48
  t/1329 -> concatenate10/49
  t/1330 -> concatenate10/50
  t/1331 -> concatenate10/51
  t/1332 -> concatenate10/52
  t/1333 -> concatenate10/53
  t/1334 -> concatenate10/54
  t/1335 -> concatenate10/55
  t/1336 -> concatenate10/56
  t/1337 -> concatenate10/57
  t/1338 -> concatenate10/58
  t/1339 -> concatenate10/59
  t/1340 -> concatenate10/60
  t/1341 -> concatenate10/61
  t/1342 -> concatenate10/62
  t/1343 -> concatenate10/63
  t/1344 -> concatenate10/64
  t/1345 -> concatenate10/65
  t/1346 -> concatenate10/66
  t/1347 -> concatenate10/67
  t/1348 -> concatenate10/68
  t/1349 -> concatenate10/69
  t/1350 -> concatenate10/70
  t/1351 -> concatenate10/71
  t/1352 -> concatenate10/72
  t/1353 -> concatenate10/73
  t/1354 -> concatenate10/74
  t/1355 -> concatenate10/75
  t/1356 -> concatenate10/76
  t/1357 -> concatenate10/77
  t/1358 -> concatenate10/78
  t/1359 -> concatenate10/79
  t/1360 -> concatenate10/80
  t/1361 -> concatenate10/81
  t/1362 -> concatenate10/82
  t/1363 -> concatenate10/83
  t/1364 -> concatenate10/84
  t/1365 -> concatenate10/85
  t/1366 -> concatenate10/86
  t/1367 -> concatenate10/87
  t/1368 -> concatenate10/88
  t/1369 -> concatenate10/89
  t/1370 -> concatenate10/90
  t/1371 -> concatenate10/91
  t/1372 -> concatenate10/92
  t/1373 -> concatenate10/93
  t/1374 -> concatenate10/94
  t/1375 -> concatenate10/95
  t/1376 -> concatenate10/96
  t/1377 -> concatenate10/97
  t/1378 -> concatenate10/98
  t/1379 -> concatenate10/99
  t/1380 -> concatenate10/100
  t/1381 -> concatenate10/101
  t/1382 -> concatenate10/102
  t/1383 -> concatenate10/103
  t/1384 -> concatenate10/104
  t/1385 -> concatenate10/105
  t/1386 -> concatenate10/106
  t/1387 -> concatenate10/107
  t/1388 -> concatenate10/108
  t/1389 -> concatenate10/109
  t/1390 -> concatenate10/110
  t/1391 -> concatenate10/111
  t/1392 -> concatenate10/112
  t/1393 -> concatenate10/113
  t/1394 -> concatenate10/114
  t/1395 -> concatenate10/115
  t/1396 -> concatenate10/116
  t/1397 -> concatenate10/117
  t/1398 -> concatenate10/118
  t/1399 -> concatenate10/119
  t/1400 -> concatenate10/120
  t/1401 -> concatenate10/121
  t/1402 -> concatenate10/122
  t/1403 -> concatenate10/123
  t/1404 -> concatenate10/124
  t/1405 -> concatenate10/125
  t/1406 -> concatenate10/126
  t/1407 -> concatenate10/127
  t/1408 -> concatenate10/128
  t/1409 -> concatenate11/1
  t/1410 -> concatenate11/2
  t/1411 -> concatenate11/3
  t/1412 -> concatenate11/4
  t/1413 -> concatenate11/5
  t/1414 -> concatenate11/6
  t/1415 -> concatenate11/7
  t/1416 -> concatenate11/8
  t/1417 -> concatenate11/9
  t/1418 -> concatenate11/10
  t/1419 -> concatenate11/11
  t/1420 -> concatenate11/12
  t/1421 -> concatenate11/13
  t/1422 -> concatenate11/14
  t/1423 -> concatenate11/15
  t/1424 -> concatenate11/16
  t/1425 -> concatenate11/17
  t/1426 -> concatenate11/18
  t/1427 -> concatenate11/19
  t/1428 -> concatenate11/20
  t/1429 -> concatenate11/21
  t/1430 -> concatenate11/22
  t/1431 -> concatenate11/23
  t/1432 -> concatenate11/24
  t/1433 -> concatenate11/25
  t/1434 -> concatenate11/26
  t/1435 -> concatenate11/27
  t/1436 -> concatenate11/28
  t/1437 -> concatenate11/29
  t/1438 -> concatenate11/30
  t/1439 -> concatenate11/31
  t/1440 -> concatenate11/32
  t/1441 -> concatenate11/33
  t/1442 -> concatenate11/34
  t/1443 -> concatenate11/35
  t/1444 -> concatenate11/36
  t/1445 -> concatenate11/37
  t/1446 -> concatenate11/38
  t/1447 -> concatenate11/39
  t/1448 -> concatenate11/40
  t/1449 -> concatenate11/41
  t/1450 -> concatenate11/42
  t/1451 -> concatenate11/43
  t/1452 -> concatenate11/44
  t/1453 -> concatenate11/45
  t/1454 -> concatenate11/46
  t/1455 -> concatenate11/47
  t/1456 -> concatenate11/48
  t/1457 -> concatenate11/49
  t/1458 -> concatenate11/50
  t/1459 -> concatenate11/51
  t/1460 -> concatenate11/52
  t/1461 -> concatenate11/53
  t/1462 -> concatenate11/54
  t/1463 -> concatenate11/55
  t/1464 -> concatenate11/56
  t/1465 -> concatenate11/57
  t/1466 -> concatenate11/58
  t/1467 -> concatenate11/59
  t/1468 -> concatenate11/60
  t/1469 -> concatenate11/61
  t/1470 -> concatenate11/62
  t/1471 -> concatenate11/63
  t/1472 -> concatenate11/64
  t/1473 -> concatenate11/65
  t/1474 -> concatenate11/66
  t/1475 -> concatenate11/67
  t/1476 -> concatenate11/68
  t/1477 -> concatenate11/69
  t/1478 -> concatenate11/70
  t/1479 -> concatenate11/71
  t/1480 -> concatenate11/72
  t/1481 -> concatenate11/73
  t/1482 -> concatenate11/74
  t/1483 -> concatenate11/75
  t/1484 -> concatenate11/76
  t/1485 -> concatenate11/77
  t/1486 -> concatenate11/78
  t/1487 -> concatenate11/79
  t/1488 -> concatenate11/80
  t/1489 -> concatenate11/81
  t/1490 -> concatenate11/82
  t/1491 -> concatenate11/83
  t/1492 -> concatenate11/84
  t/1493 -> concatenate11/85
  t/1494 -> concatenate11/86
  t/1495 -> concatenate11/87
  t/1496 -> concatenate11/88
  t/1497 -> concatenate11/89
  t/1498 -> concatenate11/90
  t/1499 -> concatenate11/91
  t/1500 -> concatenate11/92
  t/1501 -> concatenate11/93
  t/1502 -> concatenate11/94
  t/1503 -> concatenate11/95
  t/1504 -> concatenate11/96
  t/1505 -> concatenate11/97
  t/1506 -> concatenate11/98
  t/1507 -> concatenate11/99
  t/1508 -> concatenate11/100
  t/1509 -> concatenate11/101
  t/1510 -> concatenate11/102
  t/1511 -> concatenate11/103
  t/1512 -> concatenate11/104
  t/1513 -> concatenate11/105
  t/1514 -> concatenate11/106
  t/1515 -> concatenate11/107
  t/1516 -> concatenate11/108
  t/1517 -> concatenate11/109
  t/1518 -> concatenate11/110
  t/1519 -> concatenate11/111
  t/1520 -> concatenate11/112
  t/1521 -> concatenate11/113
  t/1522 -> concatenate11/114
  t/1523 -> concatenate11/115
  t/1524 -> concatenate11/116
  t/1525 -> concatenate11/117
  t/1526 -> concatenate11/118
  t/1527 -> concatenate11/119
  t/1528 -> concatenate11/120
  t/1529 -> concatenate11/121
  t/1530 -> concatenate11/122
  t/1531 -> concatenate11/123
  t/1532 -> concatenate11/124
  t/1533 -> concatenate11/125
  t/1534 -> concatenate11/126
  t/1535 -> concatenate11/127
  t/1536 -> concatenate11/128
  t/1537 -> concatenate12/1
  t/1538 -> concatenate12/2
  t/1539 -> concatenate12/3
  t/1540 -> concatenate12/4
  t/1541 -> concatenate12/5
  t/1542 -> concatenate12/6
  t/1543 -> concatenate12/7
  t/1544 -> concatenate12/8
  t/1545 -> concatenate12/9
  t/1546 -> concatenate12/10
  t/1547 -> concatenate12/11
  t/1548 -> concatenate12/12
  t/1549 -> concatenate12/13
  t/1550 -> concatenate12/14
  t/1551 -> concatenate12/15
  t/1552 -> concatenate12/16
  t/1553 -> concatenate12/17
  t/1554 -> concatenate12/18
  t/1555 -> concatenate12/19
  t/1556 -> concatenate12/20
  t/1557 -> concatenate12/21
  t/1558 -> concatenate12/22
  t/1559 -> concatenate12/23
  t/1560 -> concatenate12/24
  t/1561 -> concatenate12/25
  t/1562 -> concatenate12/26
  t/1563 -> concatenate12/27
  t/1564 -> concatenate12/28
  t/1565 -> concatenate12/29
  t/1566 -> concatenate12/30
  t/1567 -> concatenate12/31
  t/1568 -> concatenate12/32
  t/1569 -> concatenate12/33
  t/1570 -> concatenate12/34
  t/1571 -> concatenate12/35
  t/1572 -> concatenate12/36
  t/1573 -> concatenate12/37
  t/1574 -> concatenate12/38
  t/1575 -> concatenate12/39
  t/1576 -> concatenate12/40
  t/1577 -> concatenate12/41
  t/1578 -> concatenate12/42
  t/1579 -> concatenate12/43
  t/1580 -> concatenate12/44
  t/1581 -> concatenate12/45
  t/1582 -> concatenate12/46
  t/1583 -> concatenate12/47
  t/1584 -> concatenate12/48
  t/1585 -> concatenate12/49
  t/1586 -> concatenate12/50
  t/1587 -> concatenate12/51
  t/1588 -> concatenate12/52
  t/1589 -> concatenate12/53
  t/1590 -> concatenate12/54
  t/1591 -> concatenate12/55
  t/1592 -> concatenate12/56
  t/1593 -> concatenate12/57
  t/1594 -> concatenate12/58
  t/1595 -> concatenate12/59
  t/1596 -> concatenate12/60
  t/1597 -> concatenate12/61
  t/1598 -> concatenate12/62
  t/1599 -> concatenate12/63
  t/1600 -> concatenate12/64
  t/1601 -> concatenate12/65
  t/1602 -> concatenate12/66
  t/1603 -> concatenate12/67
  t/1604 -> concatenate12/68
  t/1605 -> concatenate12/69
  t/1606 -> concatenate12/70
  t/1607 -> concatenate12/71
  t/1608 -> concatenate12/72
  t/1609 -> concatenate12/73
  t/1610 -> concatenate12/74
  t/1611 -> concatenate12/75
  t/1612 -> concatenate12/76
  t/1613 -> concatenate12/77
  t/1614 -> concatenate12/78
  t/1615 -> concatenate12/79
  t/1616 -> concatenate12/80
  t/1617 -> concatenate12/81
  t/1618 -> concatenate12/82
  t/1619 -> concatenate12/83
  t/1620 -> concatenate12/84
  t/1621 -> concatenate12/85
  t/1622 -> concatenate12/86
  t/1623 -> concatenate12/87
  t/1624 -> concatenate12/88
  t/1625 -> concatenate12/89
  t/1626 -> concatenate12/90
  t/1627 -> concatenate12/91
  t/1628 -> concatenate12/92
  t/1629 -> concatenate12/93
  t/1630 -> concatenate12/94
  t/1631 -> concatenate12/95
  t/1632 -> concatenate12/96
  t/1633 -> concatenate12/97
  t/1634 -> concatenate12/98
  t/1635 -> concatenate12/99
  t/1636 -> concatenate12/100
  t/1637 -> concatenate12/101
  t/1638 -> concatenate12/102
  t/1639 -> concatenate12/103
  t/1640 -> concatenate12/104
  t/1641 -> concatenate12/105
  t/1642 -> concatenate12/106
  t/1643 -> concatenate12/107
  t/1644 -> concatenate12/108
  t/1645 -> concatenate12/109
  t/1646 -> concatenate12/110
  t/1647 -> concatenate12/111
  t/1648 -> concatenate12/112
  t/1649 -> concatenate12/113
  t/1650 -> concatenate12/114
  t/1651 -> concatenate12/115
  t/1652 -> concatenate12/116
  t/1653 -> concatenate12/117
  t/1654 -> concatenate12/118
  t/1655 -> concatenate12/119
  t/1656 -> concatenate12/120
  t/1657 -> concatenate12/121
  t/1658 -> concatenate12/122
  t/1659 -> concatenate12/123
  t/1660 -> concatenate12/124
  t/1661 -> concatenate12/125
  t/1662 -> concatenate12/126
  t/1663 -> concatenate12/127
  t/1664 -> concatenate12/128
  t/1665 -> concatenate13/1
  t/1666 -> concatenate13/2
  t/1667 -> concatenate13/3
  t/1668 -> concatenate13/4
  t/1669 -> concatenate13/5
  t/1670 -> concatenate13/6
  t/1671 -> concatenate13/7
  t/1672 -> concatenate13/8
  t/1673 -> concatenate13/9
  t/1674 -> concatenate13/10
  t/1675 -> concatenate13/11
  t/1676 -> concatenate13/12
  t/1677 -> concatenate13/13
  t/1678 -> concatenate13/14
  t/1679 -> concatenate13/15
  t/1680 -> concatenate13/16
  t/1681 -> concatenate13/17
  t/1682 -> concatenate13/18
  t/1683 -> concatenate13/19
  t/1684 -> concatenate13/20
  t/1685 -> concatenate13/21
  t/1686 -> concatenate13/22
  t/1687 -> concatenate13/23
  t/1688 -> concatenate13/24
  t/1689 -> concatenate13/25
  t/1690 -> concatenate13/26
  t/1691 -> concatenate13/27
  t/1692 -> concatenate13/28
  t/1693 -> concatenate13/29
  t/1694 -> concatenate13/30
  t/1695 -> concatenate13/31
  t/1696 -> concatenate13/32
  t/1697 -> concatenate13/33
  t/1698 -> concatenate13/34
  t/1699 -> concatenate13/35
  t/1700 -> concatenate13/36
  t/1701 -> concatenate13/37
  t/1702 -> concatenate13/38
  t/1703 -> concatenate13/39
  t/1704 -> concatenate13/40
  t/1705 -> concatenate13/41
  t/1706 -> concatenate13/42
  t/1707 -> concatenate13/43
  t/1708 -> concatenate13/44
  t/1709 -> concatenate13/45
  t/1710 -> concatenate13/46
  t/1711 -> concatenate13/47
  t/1712 -> concatenate13/48
  t/1713 -> concatenate13/49
  t/1714 -> concatenate13/50
  t/1715 -> concatenate13/51
  t/1716 -> concatenate13/52
  t/1717 -> concatenate13/53
  t/1718 -> concatenate13/54
  t/1719 -> concatenate13/55
  t/1720 -> concatenate13/56
  t/1721 -> concatenate13/57
  t/1722 -> concatenate13/58
  t/1723 -> concatenate13/59
  t/1724 -> concatenate13/60
  t/1725 -> concatenate13/61
  t/1726 -> concatenate13/62
  t/1727 -> concatenate13/63
  t/1728 -> concatenate13/64
  t/1729 -> concatenate13/65
  t/1730 -> concatenate13/66
  t/1731 -> concatenate13/67
  t/1732 -> concatenate13/68
  t/1733 -> concatenate13/69
  t/1734 -> concatenate13/70
  t/1735 -> concatenate13/71
  t/1736 -> concatenate13/72
  t/1737 -> concatenate13/73
  t/1738 -> concatenate13/74
  t/1739 -> concatenate13/75
  t/1740 -> concatenate13/76
  t/1741 -> concatenate13/77
  t/1742 -> concatenate13/78
  t/1743 -> concatenate13/79
  t/1744 -> concatenate13/80
  t/1745 -> concatenate13/81
  t/1746 -> concatenate13/82
  t/1747 -> concatenate13/83
  t/1748 -> concatenate13/84
  t/1749 -> concatenate13/85
  t/1750 -> concatenate13/86
  t/1751 -> concatenate13/87
  t/1752 -> concatenate13/88
  t/1753 -> concatenate13/89
  t/1754 -> concatenate13/90
  t/1755 -> concatenate13/91
  t/1756 -> concatenate13/92
  t/1757 -> concatenate13/93
  t/1758 -> concatenate13/94
  t/1759 -> concatenate13/95
  t/1760 -> concatenate13/96
  t/1761 -> concatenate13/97
  t/1762 -> concatenate13/98
  t/1763 -> concatenate13/99
  t/1764 -> concatenate13/100
  t/1765 -> concatenate13/101
  t/1766 -> concatenate13/102
  t/1767 -> concatenate13/103
  t/1768 -> concatenate13/104
  t/1769 -> concatenate13/105
  t/1770 -> concatenate13/106
  t/1771 -> concatenate13/107
  t/1772 -> concatenate13/108
  t/1773 -> concatenate13/109
  t/1774 -> concatenate13/110
  t/1775 -> concatenate13/111
  t/1776 -> concatenate13/112
  t/1777 -> concatenate13/113
  t/1778 -> concatenate13/114
  t/1779 -> concatenate13/115
  t/1780 -> concatenate13/116
  t/1781 -> concatenate13/117
  t/1782 -> concatenate13/118
  t/1783 -> concatenate13/119
  t/1784 -> concatenate13/120
  t/1785 -> concatenate13/121
  t/1786 -> concatenate13/122
  t/1787 -> concatenate13/123
  t/1788 -> concatenate13/124
  t/1789 -> concatenate13/125
  t/1790 -> concatenate13/126
  t/1791 -> concatenate13/127
  t/1792 -> concatenate13/128
  t/1793 -> concatenate14/1
  t/1794 -> concatenate14/2
  t/1795 -> concatenate14/3
  t/1796 -> concatenate14/4
  t/1797 -> concatenate14/5
  t/1798 -> concatenate14/6
  t/1799 -> concatenate14/7
  t/1800 -> concatenate14/8
  t/1801 -> concatenate14/9
  t/1802 -> concatenate14/10
  t/1803 -> concatenate14/11
  t/1804 -> concatenate14/12
  t/1805 -> concatenate14/13
  t/1806 -> concatenate14/14
  t/1807 -> concatenate14/15
  t/1808 -> concatenate14/16
  t/1809 -> concatenate14/17
  t/1810 -> concatenate14/18
  t/1811 -> concatenate14/19
  t/1812 -> concatenate14/20
  t/1813 -> concatenate14/21
  t/1814 -> concatenate14/22
  t/1815 -> concatenate14/23
  t/1816 -> concatenate14/24
  t/1817 -> concatenate14/25
  t/1818 -> concatenate14/26
  t/1819 -> concatenate14/27
  t/1820 -> concatenate14/28
  t/1821 -> concatenate14/29
  t/1822 -> concatenate14/30
  t/1823 -> concatenate14/31
  t/1824 -> concatenate14/32
  t/1825 -> concatenate14/33
  t/1826 -> concatenate14/34
  t/1827 -> concatenate14/35
  t/1828 -> concatenate14/36
  t/1829 -> concatenate14/37
  t/1830 -> concatenate14/38
  t/1831 -> concatenate14/39
  t/1832 -> concatenate14/40
  t/1833 -> concatenate14/41
  t/1834 -> concatenate14/42
  t/1835 -> concatenate14/43
  t/1836 -> concatenate14/44
  t/1837 -> concatenate14/45
  t/1838 -> concatenate14/46
  t/1839 -> concatenate14/47
  t/1840 -> concatenate14/48
  t/1841 -> concatenate14/49
  t/1842 -> concatenate14/50
  t/1843 -> concatenate14/51
  t/1844 -> concatenate14/52
  t/1845 -> concatenate14/53
  t/1846 -> concatenate14/54
  t/1847 -> concatenate14/55
  t/1848 -> concatenate14/56
  t/1849 -> concatenate14/57
  t/1850 -> concatenate14/58
  t/1851 -> concatenate14/59
  t/1852 -> concatenate14/60
  t/1853 -> concatenate14/61
  t/1854 -> concatenate14/62
  t/1855 -> concatenate14/63
  t/1856 -> concatenate14/64
  t/1857 -> concatenate14/65
  t/1858 -> concatenate14/66
  t/1859 -> concatenate14/67
  t/1860 -> concatenate14/68
  t/1861 -> concatenate14/69
  t/1862 -> concatenate14/70
  t/1863 -> concatenate14/71
  t/1864 -> concatenate14/72
  t/1865 -> concatenate14/73
  t/1866 -> concatenate14/74
  t/1867 -> concatenate14/75
  t/1868 -> concatenate14/76
  t/1869 -> concatenate14/77
  t/1870 -> concatenate14/78
  t/1871 -> concatenate14/79
  t/1872 -> concatenate14/80
  t/1873 -> concatenate14/81
  t/1874 -> concatenate14/82
  t/1875 -> concatenate14/83
  t/1876 -> concatenate14/84
  t/1877 -> concatenate14/85
  t/1878 -> concatenate14/86
  t/1879 -> concatenate14/87
  t/1880 -> concatenate14/88
  t/1881 -> concatenate14/89
  t/1882 -> concatenate14/90
  t/1883 -> concatenate14/91
  t/1884 -> concatenate14/92
  t/1885 -> concatenate14/93
  t/1886 -> concatenate14/94
  t/1887 -> concatenate14/95
  t/1888 -> concatenate14/96
  t/1889 -> concatenate14/97
  t/1890 -> concatenate14/98
  t/1891 -> concatenate14/99
  t/1892 -> concatenate14/100
  t/1893 -> concatenate14/101
  t/1894 -> concatenate14/102
  t/1895 -> concatenate14/103
  t/1896 -> concatenate14/104
  t/1897 -> concatenate14/105
  t/1898 -> concatenate14/106
  t/1899 -> concatenate14/107
  t/1900 -> concatenate14/108
  t/1901 -> concatenate14/109
  t/1902 -> concatenate14/110
  t/1903 -> concatenate14/111
  t/1904 -> concatenate14/112
  t/1905 -> concatenate14/113
  t/1906 -> concatenate14/114
  t/1907 -> concatenate14/115
  t/1908 -> concatenate14/116
  t/1909 -> concatenate14/117
  t/1910 -> concatenate14/118
  t/1911 -> concatenate14/119
  t/1912 -> concatenate14/120
  t/1913 -> concatenate14/121
  t/1914 -> concatenate14/122
  t/1915 -> concatenate14/123
  t/1916 -> concatenate14/124
  t/1917 -> concatenate14/125
  t/1918 -> concatenate14/126
  t/1919 -> concatenate14/127
  t/1920 -> concatenate14/128
  t/1921 -> concatenate15/1
  t/1922 -> concatenate15/2
  t/1923 -> concatenate15/3
  t/1924 -> concatenate15/4
  t/1925 -> concatenate15/5
  t/1926 -> concatenate15/6
  t/1927 -> concatenate15/7
  t/1928 -> concatenate15/8
  t/1929 -> concatenate15/9
  t/1930 -> concatenate15/10
  t/1931 -> concatenate15/11
  t/1932 -> concatenate15/12
  t/1933 -> concatenate15/13
  t/1934 -> concatenate15/14
  t/1935 -> concatenate15/15
  t/1936 -> concatenate15/16
  t/1937 -> concatenate15/17
  t/1938 -> concatenate15/18
  t/1939 -> concatenate15/19
  t/1940 -> concatenate15/20
  t/1941 -> concatenate15/21
  t/1942 -> concatenate15/22
  t/1943 -> concatenate15/23
  t/1944 -> concatenate15/24
  t/1945 -> concatenate15/25
  t/1946 -> concatenate15/26
  t/1947 -> concatenate15/27
  t/1948 -> concatenate15/28
  t/1949 -> concatenate15/29
  t/1950 -> concatenate15/30
  t/1951 -> concatenate15/31
  t/1952 -> concatenate15/32
  t/1953 -> concatenate15/33
  t/1954 -> concatenate15/34
  t/1955 -> concatenate15/35
  t/1956 -> concatenate15/36
  t/1957 -> concatenate15/37
  t/1958 -> concatenate15/38
  t/1959 -> concatenate15/39
  t/1960 -> concatenate15/40
  t/1961 -> concatenate15/41
  t/1962 -> concatenate15/42
  t/1963 -> concatenate15/43
  t/1964 -> concatenate15/44
  t/1965 -> concatenate15/45
  t/1966 -> concatenate15/46
  t/1967 -> concatenate15/47
  t/1968 -> concatenate15/48
  t/1969 -> concatenate15/49
  t/1970 -> concatenate15/50
  t/1971 -> concatenate15/51
  t/1972 -> concatenate15/52
  t/1973 -> concatenate15/53
  t/1974 -> concatenate15/54
  t/1975 -> concatenate15/55
  t/1976 -> concatenate15/56
  t/1977 -> concatenate15/57
  t/1978 -> concatenate15/58
  t/1979 -> concatenate15/59
  t/1980 -> concatenate15/60
  t/1981 -> concatenate15/61
  t/1982 -> concatenate15/62
  t/1983 -> concatenate15/63
  t/1984 -> concatenate15/64
  t/1985 -> concatenate15/65
  t/1986 -> concatenate15/66
  t/1987 -> concatenate15/67
  t/1988 -> concatenate15/68
  t/1989 -> concatenate15/69
  t/1990 -> concatenate15/70
  t/1991 -> concatenate15/71
  t/1992 -> concatenate15/72
  t/1993 -> concatenate15/73
  t/1994 -> concatenate15/74
  t/1995 -> concatenate15/75
  t/1996 -> concatenate15/76
  t/1997 -> concatenate15/77
  t/1998 -> concatenate15/78
  t/1999 -> concatenate15/79
  t/2000 -> concatenate15/80
  t/2001 -> concatenate15/81
  t/2002 -> concatenate15/82
  t/2003 -> concatenate15/83
  t/2004 -> concatenate15/84
  t/2005 -> concatenate15/85
  t/2006 -> concatenate15/86
  t/2007 -> concatenate15/87
  t/2008 -> concatenate15/88
  t/2009 -> concatenate15/89
  t/2010 -> concatenate15/90
  t/2011 -> concatenate15/91
  t/2012 -> concatenate15/92
  t/2013 -> concatenate15/93
  t/2014 -> concatenate15/94
  t/2015 -> concatenate15/95
  t/2016 -> concatenate15/96
  t/2017 -> concatenate15/97
  t/2018 -> concatenate15/98
  t/2019 -> concatenate15/99
  t/2020 -> concatenate15/100
  t/2021 -> concatenate15/101
  t/2022 -> concatenate15/102
  t/2023 -> concatenate15/103
  t/2024 -> concatenate15/104
  t/2025 -> concatenate15/105
  t/2026 -> concatenate15/106
  t/2027 -> concatenate15/107
  t/2028 -> concatenate15/108
  t/2029 -> concatenate15/109
  t/2030 -> concatenate15/110
  t/2031 -> concatenate15/111
  t/2032 -> concatenate15/112
  t/2033 -> concatenate15/113
  t/2034 -> concatenate15/114
  t/2035 -> concatenate15/115
  t/2036 -> concatenate15/116
  t/2037 -> concatenate15/117
  t/2038 -> concatenate15/118
  t/2039 -> concatenate15/119
  t/2040 -> concatenate15/120
  t/2041 -> concatenate15/121
  t/2042 -> concatenate15/122
  t/2043 -> concatenate15/123
  t/2044 -> concatenate15/124
  t/2045 -> concatenate15/125
  t/2046 -> concatenate15/126
  t/2047 -> concatenate15/127
  t/2048 -> concatenate15/128
  t/2049 -> concatenate16/1
  t/2050 -> concatenate16/2
  t/2051 -> concatenate16/3
  t/2052 -> concatenate16/4
  t/2053 -> concatenate16/5
  t/2054 -> concatenate16/6
  t/2055 -> concatenate16/7
  t/2056 -> concatenate16/8
  t/2057 -> concatenate16/9
  t/2058 -> concatenate16/10
  t/2059 -> concatenate16/11
  t/2060 -> concatenate16/12
  t/2061 -> concatenate16/13
  t/2062 -> concatenate16/14
  t/2063 -> concatenate16/15
  t/2064 -> concatenate16/16
  t/2065 -> concatenate16/17
  t/2066 -> concatenate16/18
  t/2067 -> concatenate16/19
  t/2068 -> concatenate16/20
  t/2069 -> concatenate16/21
  t/2070 -> concatenate16/22
  t/2071 -> concatenate16/23
  t/2072 -> concatenate16/24
  t/2073 -> concatenate16/25
  t/2074 -> concatenate16/26
  t/2075 -> concatenate16/27
  t/2076 -> concatenate16/28
  t/2077 -> concatenate16/29
  t/2078 -> concatenate16/30
  t/2079 -> concatenate16/31
  t/2080 -> concatenate16/32
  t/2081 -> concatenate16/33
  t/2082 -> concatenate16/34
  t/2083 -> concatenate16/35
  t/2084 -> concatenate16/36
  t/2085 -> concatenate16/37
  t/2086 -> concatenate16/38
  t/2087 -> concatenate16/39
  t/2088 -> concatenate16/40
  t/2089 -> concatenate16/41
  t/2090 -> concatenate16/42
  t/2091 -> concatenate16/43
  t/2092 -> concatenate16/44
  t/2093 -> concatenate16/45
  t/2094 -> concatenate16/46
  t/2095 -> concatenate16/47
  t/2096 -> concatenate16/48
  t/2097 -> concatenate16/49
  t/2098 -> concatenate16/50
  t/2099 -> concatenate16/51
  t/2100 -> concatenate16/52
  t/2101 -> concatenate16/53
  t/2102 -> concatenate16/54
  t/2103 -> concatenate16/55
  t/2104 -> concatenate16/56
  t/2105 -> concatenate16/57
  t/2106 -> concatenate16/58
  t/2107 -> concatenate16/59
  t/2108 -> concatenate16/60
  t/2109 -> concatenate16/61
  t/2110 -> concatenate16/62
  t/2111 -> concatenate16/63
  t/2112 -> concatenate16/64
  t/2113 -> concatenate16/65
  t/2114 -> concatenate16/66
  t/2115 -> concatenate16/67
  t/2116 -> concatenate16/68
  t/2117 -> concatenate16/69
  t/2118 -> concatenate16/70
  t/2119 -> concatenate16/71
  t/2120 -> concatenate16/72
  t/2121 -> concatenate16/73
  t/2122 -> concatenate16/74
  t/2123 -> concatenate16/75
  t/2124 -> concatenate16/76
  t/2125 -> concatenate16/77
  t/2126 -> concatenate16/78
  t/2127 -> concatenate16/79
  t/2128 -> concatenate16/80
  t/2129 -> concatenate16/81
  t/2130 -> concatenate16/82
  t/2131 -> concatenate16/83
  t/2132 -> concatenate16/84
  t/2133 -> concatenate16/85
  t/2134 -> concatenate16/86
  t/2135 -> concatenate16/87
  t/2136 -> concatenate16/88
  t/2137 -> concatenate16/89
  t/2138 -> concatenate16/90
  t/2139 -> concatenate16/91
  t/2140 -> concatenate16/92
  t/2141 -> concatenate16/93
  t/2142 -> concatenate16/94
  t/2143 -> concatenate16/95
  t/2144 -> concatenate16/96
  t/2145 -> concatenate16/97
  t/2146 -> concatenate16/98
  t/2147 -> concatenate16/99
  t/2148 -> concatenate16/100
  t/2149 -> concatenate16/101
  t/2150 -> concatenate16/102
  t/2151 -> concatenate16/103
  t/2152 -> concatenate16/104
  t/2153 -> concatenate16/105
  t/2154 -> concatenate16/106
  t/2155 -> concatenate16/107
  t/2156 -> concatenate16/108
  t/2157 -> concatenate16/109
  t/2158 -> concatenate16/110
  t/2159 -> concatenate16/111
  t/2160 -> concatenate16/112
  t/2161 -> concatenate16/113
  t/2162 -> concatenate16/114
  t/2163 -> concatenate16/115
  t/2164 -> concatenate16/116
  t/2165 -> concatenate16/117
  t/2166 -> concatenate16/118
  t/2167 -> concatenate16/119
  t/2168 -> concatenate16/120
  t/2169 -> concatenate16/121
  t/2170 -> concatenate16/122
  t/2171 -> concatenate16/123
  t/2172 -> concatenate16/124
  t/2173 -> concatenate16/125
  t/2174 -> concatenate16/126
  t/2175 -> concatenate16/127
  t/2176 -> concatenate16/128
  t/2177 -> concatenate17/1
  t/2178 -> concatenate17/2
  t/2179 -> concatenate17/3
  t/2180 -> concatenate17/4
  t/2181 -> concatenate17/5
  t/2182 -> concatenate17/6
  t/2183 -> concatenate17/7
  t/2184 -> concatenate17/8
  t/2185 -> concatenate17/9
  t/2186 -> concatenate17/10
  t/2187 -> concatenate17/11
  t/2188 -> concatenate17/12
  t/2189 -> concatenate17/13
  t/2190 -> concatenate17/14
  t/2191 -> concatenate17/15
  t/2192 -> concatenate17/16
  t/2193 -> concatenate17/17
  t/2194 -> concatenate17/18
  t/2195 -> concatenate17/19
  t/2196 -> concatenate17/20
  t/2197 -> concatenate17/21
  t/2198 -> concatenate17/22
  t/2199 -> concatenate17/23
  t/2200 -> concatenate17/24
  t/2201 -> concatenate17/25
  t/2202 -> concatenate17/26
  t/2203 -> concatenate17/27
  t/2204 -> concatenate17/28
  t/2205 -> concatenate17/29
  t/2206 -> concatenate17/30
  t/2207 -> concatenate17/31
  t/2208 -> concatenate17/32
  t/2209 -> concatenate17/33
  t/2210 -> concatenate17/34
  t/2211 -> concatenate17/35
  t/2212 -> concatenate17/36
  t/2213 -> concatenate17/37
  t/2214 -> concatenate17/38
  t/2215 -> concatenate17/39
  t/2216 -> concatenate17/40
  t/2217 -> concatenate17/41
  t/2218 -> concatenate17/42
  t/2219 -> concatenate17/43
  t/2220 -> concatenate17/44
  t/2221 -> concatenate17/45
  t/2222 -> concatenate17/46
  t/2223 -> concatenate17/47
  t/2224 -> concatenate17/48
  t/2225 -> concatenate17/49
  t/2226 -> concatenate17/50
  t/2227 -> concatenate17/51
  t/2228 -> concatenate17/52
  t/2229 -> concatenate17/53
  t/2230 -> concatenate17/54
  t/2231 -> concatenate17/55
  t/2232 -> concatenate17/56
  t/2233 -> concatenate17/57
  t/2234 -> concatenate17/58
  t/2235 -> concatenate17/59
  t/2236 -> concatenate17/60
  t/2237 -> concatenate17/61
  t/2238 -> concatenate17/62
  t/2239 -> concatenate17/63
  t/2240 -> concatenate17/64
  t/2241 -> concatenate17/65
  t/2242 -> concatenate17/66
  t/2243 -> concatenate17/67
  t/2244 -> concatenate17/68
  t/2245 -> concatenate17/69
  t/2246 -> concatenate17/70
  t/2247 -> concatenate17/71
  t/2248 -> concatenate17/72
  t/2249 -> concatenate17/73
  t/2250 -> concatenate17/74
  t/2251 -> concatenate17/75
  t/2252 -> concatenate17/76
  t/2253 -> concatenate17/77
  t/2254 -> concatenate17/78
  t/2255 -> concatenate17/79
  t/2256 -> concatenate17/80
  t/2257 -> concatenate17/81
  t/2258 -> concatenate17/82
  t/2259 -> concatenate17/83
  t/2260 -> concatenate17/84
  t/2261 -> concatenate17/85
  t/2262 -> concatenate17/86
  t/2263 -> concatenate17/87
  t/2264 -> concatenate17/88
  t/2265 -> concatenate17/89
  t/2266 -> concatenate17/90
  t/2267 -> concatenate17/91
  t/2268 -> concatenate17/92
  t/2269 -> concatenate17/93
  t/2270 -> concatenate17/94
  t/2271 -> concatenate17/95
  t/2272 -> concatenate17/96
  t/2273 -> concatenate17/97
  t/2274 -> concatenate17/98
  t/2275 -> concatenate17/99
  t/2276 -> concatenate17/100
  t/2277 -> concatenate17/101
  t/2278 -> concatenate17/102
  t/2279 -> concatenate17/103
  t/2280 -> concatenate17/104
  t/2281 -> concatenate17/105
  t/2282 -> concatenate17/106
  t/2283 -> concatenate17/107
  t/2284 -> concatenate17/108
  t/2285 -> concatenate17/109
  t/2286 -> concatenate17/110
  t/2287 -> concatenate17/111
  t/2288 -> concatenate17/112
  t/2289 -> concatenate17/113
  t/2290 -> concatenate17/114
  t/2291 -> concatenate17/115
  t/2292 -> concatenate17/116
  t/2293 -> concatenate17/117
  t/2294 -> concatenate17/118
  t/2295 -> concatenate17/119
  t/2296 -> concatenate17/120
  t/2297 -> concatenate17/121
  t/2298 -> concatenate17/122
  t/2299 -> concatenate17/123
  t/2300 -> concatenate17/124
  t/2301 -> concatenate17/125
  t/2302 -> concatenate17/126
  t/2303 -> concatenate17/127
  t/2304 -> concatenate17/128
  t/2305 -> concatenate18/1
  t/2306 -> concatenate18/2
  t/2307 -> concatenate18/3
  t/2308 -> concatenate18/4
  t/2309 -> concatenate18/5
  t/2310 -> concatenate18/6
  t/2311 -> concatenate18/7
  t/2312 -> concatenate18/8
  t/2313 -> concatenate18/9
  t/2314 -> concatenate18/10
  t/2315 -> concatenate18/11
  t/2316 -> concatenate18/12
  t/2317 -> concatenate18/13
  t/2318 -> concatenate18/14
  t/2319 -> concatenate18/15
  t/2320 -> concatenate18/16
  t/2321 -> concatenate18/17
  t/2322 -> concatenate18/18
  t/2323 -> concatenate18/19
  t/2324 -> concatenate18/20
  t/2325 -> concatenate18/21
  t/2326 -> concatenate18/22
  t/2327 -> concatenate18/23
  t/2328 -> concatenate18/24
  t/2329 -> concatenate18/25
  t/2330 -> concatenate18/26
  t/2331 -> concatenate18/27
  t/2332 -> concatenate18/28
  t/2333 -> concatenate18/29
  t/2334 -> concatenate18/30
  t/2335 -> concatenate18/31
  t/2336 -> concatenate18/32
  t/2337 -> concatenate18/33
  t/2338 -> concatenate18/34
  t/2339 -> concatenate18/35
  t/2340 -> concatenate18/36
  t/2341 -> concatenate18/37
  t/2342 -> concatenate18/38
  t/2343 -> concatenate18/39
  t/2344 -> concatenate18/40
  t/2345 -> concatenate18/41
  t/2346 -> concatenate18/42
  t/2347 -> concatenate18/43
  t/2348 -> concatenate18/44
  t/2349 -> concatenate18/45
  t/2350 -> concatenate18/46
  t/2351 -> concatenate18/47
  t/2352 -> concatenate18/48
  t/2353 -> concatenate18/49
  t/2354 -> concatenate18/50
  t/2355 -> concatenate18/51
  t/2356 -> concatenate18/52
  t/2357 -> concatenate18/53
  t/2358 -> concatenate18/54
  t/2359 -> concatenate18/55
  t/2360 -> concatenate18/56
  t/2361 -> concatenate18/57
  t/2362 -> concatenate18/58
  t/2363 -> concatenate18/59
  t/2364 -> concatenate18/60
  t/2365 -> concatenate18/61
  t/2366 -> concatenate18/62
  t/2367 -> concatenate18/63
  t/2368 -> concatenate18/64
  t/2369 -> concatenate18/65
  t/2370 -> concatenate18/66
  t/2371 -> concatenate18/67
  t/2372 -> concatenate18/68
  t/2373 -> concatenate18/69
  t/2374 -> concatenate18/70
  t/2375 -> concatenate18/71
  t/2376 -> concatenate18/72
  t/2377 -> concatenate18/73
  t/2378 -> concatenate18/74
  t/2379 -> concatenate18/75
  t/2380 -> concatenate18/76
  t/2381 -> concatenate18/77
  t/2382 -> concatenate18/78
  t/2383 -> concatenate18/79
  t/2384 -> concatenate18/80
  t/2385 -> concatenate18/81
  t/2386 -> concatenate18/82
  t/2387 -> concatenate18/83
  t/2388 -> concatenate18/84
  t/2389 -> concatenate18/85
  t/2390 -> concatenate18/86
  t/2391 -> concatenate18/87
  t/2392 -> concatenate18/88
  t/2393 -> concatenate18/89
  t/2394 -> concatenate18/90
  t/2395 -> concatenate18/91
  t/2396 -> concatenate18/92
  t/2397 -> concatenate18/93
  t/2398 -> concatenate18/94
  t/2399 -> concatenate18/95
  t/2400 -> concatenate18/96
  t/2401 -> concatenate18/97
  t/2402 -> concatenate18/98
  t/2403 -> concatenate18/99
  t/2404 -> concatenate18/100
  t/2405 -> concatenate18/101
  t/2406 -> concatenate18/102
  t/2407 -> concatenate18/103
  t/2408 -> concatenate18/104
  t/2409 -> concatenate18/105
  t/2410 -> concatenate18/106
  t/2411 -> concatenate18/107
  t/2412 -> concatenate18/108
  t/2413 -> concatenate18/109
  t/2414 -> concatenate18/110
  t/2415 -> concatenate18/111
  t/2416 -> concatenate18/112
  t/2417 -> concatenate18/113
  t/2418 -> concatenate18/114
  t/2419 -> concatenate18/115
  t/2420 -> concatenate18/116
  t/2421 -> concatenate18/117
  t/2422 -> concatenate18/118
  t/2423 -> concatenate18/119
  t/2424 -> concatenate18/120
  t/2425 -> concatenate18/121
  t/2426 -> concatenate18/122
  t/2427 -> concatenate18/123
  t/2428 -> concatenate18/124
  t/2429 -> concatenate18/125
  t/2430 -> concatenate18/126
  t/2431 -> concatenate18/127
  t/2432 -> concatenate18/128
  t/2433 -> concatenate19/1
  t/2434 -> concatenate19/2
  t/2435 -> concatenate19/3
  t/2436 -> concatenate19/4
  t/2437 -> concatenate19/5
  t/2438 -> concatenate19/6
  t/2439 -> concatenate19/7
  t/2440 -> concatenate19/8
  t/2441 -> concatenate19/9
  t/2442 -> concatenate19/10
  t/2443 -> concatenate19/11
  t/2444 -> concatenate19/12
  t/2445 -> concatenate19/13
  t/2446 -> concatenate19/14
  t/2447 -> concatenate19/15
  t/2448 -> concatenate19/16
  t/2449 -> concatenate19/17
  t/2450 -> concatenate19/18
  t/2451 -> concatenate19/19
  t/2452 -> concatenate19/20
  t/2453 -> concatenate19/21
  t/2454 -> concatenate19/22
  t/2455 -> concatenate19/23
  t/2456 -> concatenate19/24
  t/2457 -> concatenate19/25
  t/2458 -> concatenate19/26
  t/2459 -> concatenate19/27
  t/2460 -> concatenate19/28
  t/2461 -> concatenate19/29
  t/2462 -> concatenate19/30
  t/2463 -> concatenate19/31
  t/2464 -> concatenate19/32
  t/2465 -> concatenate19/33
  t/2466 -> concatenate19/34
  t/2467 -> concatenate19/35
  t/2468 -> concatenate19/36
  t/2469 -> concatenate19/37
  t/2470 -> concatenate19/38
  t/2471 -> concatenate19/39
  t/2472 -> concatenate19/40
  t/2473 -> concatenate19/41
  t/2474 -> concatenate19/42
  t/2475 -> concatenate19/43
  t/2476 -> concatenate19/44
  t/2477 -> concatenate19/45
  t/2478 -> concatenate19/46
  t/2479 -> concatenate19/47
  t/2480 -> concatenate19/48
  t/2481 -> concatenate19/49
  t/2482 -> concatenate19/50
  t/2483 -> concatenate19/51
  t/2484 -> concatenate19/52
  t/2485 -> concatenate19/53
  t/2486 -> concatenate19/54
  t/2487 -> concatenate19/55
  t/2488 -> concatenate19/56
  t/2489 -> concatenate19/57
  t/2490 -> concatenate19/58
  t/2491 -> concatenate19/59
  t/2492 -> concatenate19/60
  t/2493 -> concatenate19/61
  t/2494 -> concatenate19/62
  t/2495 -> concatenate19/63
  t/2496 -> concatenate19/64
  t/2497 -> concatenate19/65
  t/2498 -> concatenate19/66
  t/2499 -> concatenate19/67
  t/2500 -> concatenate19/68
  t/2501 -> concatenate19/69
  t/2502 -> concatenate19/70
  t/2503 -> concatenate19/71
  t/2504 -> concatenate19/72
  t/2505 -> concatenate19/73
  t/2506 -> concatenate19/74
  t/2507 -> concatenate19/75
  t/2508 -> concatenate19/76
  t/2509 -> concatenate19/77
  t/2510 -> concatenate19/78
  t/2511 -> concatenate19/79
  t/2512 -> concatenate19/80
  t/2513 -> concatenate19/81
  t/2514 -> concatenate19/82
  t/2515 -> concatenate19/83
  t/2516 -> concatenate19/84
  t/2517 -> concatenate19/85
  t/2518 -> concatenate19/86
  t/2519 -> concatenate19/87
  t/2520 -> concatenate19/88
  t/2521 -> concatenate19/89
  t/2522 -> concatenate19/90
  t/2523 -> concatenate19/91
  t/2524 -> concatenate19/92
  t/2525 -> concatenate19/93
  t/2526 -> concatenate19/94
  t/2527 -> concatenate19/95
  t/2528 -> concatenate19/96
  t/2529 -> concatenate19/97
  t/2530 -> concatenate19/98
  t/2531 -> concatenate19/99
  t/2532 -> concatenate19/100
  t/2533 -> concatenate19/101
  t/2534 -> concatenate19/102
  t/2535 -> concatenate19/103
  t/2536 -> concatenate19/104
  t/2537 -> concatenate19/105
  t/2538 -> concatenate19/106
  t/2539 -> concatenate19/107
  t/2540 -> concatenate19/108
  t/2541 -> concatenate19/109
  t/2542 -> concatenate19/110
  t/2543 -> concatenate19/111
  t/2544 -> concatenate19/112
  t/2545 -> concatenate19/113
  t/2546 -> concatenate19/114
  t/2547 -> concatenate19/115
  t/2548 -> concatenate19/116
  t/2549 -> concatenate19/117
  t/2550 -> concatenate19/118
  t/2551 -> concatenate19/119
  t/2552 -> concatenate19/120
  t/2553 -> concatenate19/121
  t/2554 -> concatenate19/122
  t/2555 -> concatenate19/123
  t/2556 -> concatenate19/124
  t/2557 -> concatenate19/125
  t/2558 -> concatenate19/126
  t/2559 -> concatenate19/127
  t/2560 -> concatenate19/128
  t/2561 -> concatenate20/1
  t/2562 -> concatenate20/2
  t/2563 -> concatenate20/3
  t/2564 -> concatenate20/4
  t/2565 -> concatenate20/5
  t/2566 -> concatenate20/6
  t/2567 -> concatenate20/7
  t/2568 -> concatenate20/8
  t/2569 -> concatenate20/9
  t/2570 -> concatenate20/10
  t/2571 -> concatenate20/11
  t/2572 -> concatenate20/12
  t/2573 -> concatenate20/13
  t/2574 -> concatenate20/14
  t/2575 -> concatenate20/15
  t/2576 -> concatenate20/16
  t/2577 -> concatenate20/17
  t/2578 -> concatenate20/18
  t/2579 -> concatenate20/19
  t/2580 -> concatenate20/20
  t/2581 -> concatenate20/21
  t/2582 -> concatenate20/22
  t/2583 -> concatenate20/23
  t/2584 -> concatenate20/24
  t/2585 -> concatenate20/25
  t/2586 -> concatenate20/26
  t/2587 -> concatenate20/27
  t/2588 -> concatenate20/28
  t/2589 -> concatenate20/29
  t/2590 -> concatenate20/30
  t/2591 -> concatenate20/31
  t/2592 -> concatenate20/32
  t/2593 -> concatenate20/33
  t/2594 -> concatenate20/34
  t/2595 -> concatenate20/35
  t/2596 -> concatenate20/36
  t/2597 -> concatenate20/37
  t/2598 -> concatenate20/38
  t/2599 -> concatenate20/39
  t/2600 -> concatenate20/40
  t/2601 -> concatenate20/41
  t/2602 -> concatenate20/42
  t/2603 -> concatenate20/43
  t/2604 -> concatenate20/44
  t/2605 -> concatenate20/45
  t/2606 -> concatenate20/46
  t/2607 -> concatenate20/47
  t/2608 -> concatenate20/48
  t/2609 -> concatenate20/49
  t/2610 -> concatenate20/50
  t/2611 -> concatenate20/51
  t/2612 -> concatenate20/52
  t/2613 -> concatenate20/53
  t/2614 -> concatenate20/54
  t/2615 -> concatenate20/55
  t/2616 -> concatenate20/56
  t/2617 -> concatenate20/57
  t/2618 -> concatenate20/58
  t/2619 -> concatenate20/59
  t/2620 -> concatenate20/60
  t/2621 -> concatenate20/61
  t/2622 -> concatenate20/62
  t/2623 -> concatenate20/63
  t/2624 -> concatenate20/64
  t/2625 -> concatenate20/65
  t/2626 -> concatenate20/66
  t/2627 -> concatenate20/67
  t/2628 -> concatenate20/68
  t/2629 -> concatenate20/69
  t/2630 -> concatenate20/70
  t/2631 -> concatenate20/71
  t/2632 -> concatenate20/72
  t/2633 -> concatenate20/73
  t/2634 -> concatenate20/74
  t/2635 -> concatenate20/75
  t/2636 -> concatenate20/76
  t/2637 -> concatenate20/77
  t/2638 -> concatenate20/78
  t/2639 -> concatenate20/79
  t/2640 -> concatenate20/80
  t/2641 -> concatenate20/81
  t/2642 -> concatenate20/82
  t/2643 -> concatenate20/83
  t/2644 -> concatenate20/84
  t/2645 -> concatenate20/85
  t/2646 -> concatenate20/86
  t/2647 -> concatenate20/87
  t/2648 -> concatenate20/88
  t/2649 -> concatenate20/89
  t/2650 -> concatenate20/90
  t/2651 -> concatenate20/91
  t/2652 -> concatenate20/92
  t/2653 -> concatenate20/93
  t/2654 -> concatenate20/94
  t/2655 -> concatenate20/95
  t/2656 -> concatenate20/96
  t/2657 -> concatenate20/97
  t/2658 -> concatenate20/98
  t/2659 -> concatenate20/99
  t/2660 -> concatenate20/100
  t/2661 -> concatenate20/101
  t/2662 -> concatenate20/102
  t/2663 -> concatenate20/103
  t/2664 -> concatenate20/104
  t/2665 -> concatenate20/105
  t/2666 -> concatenate20/106
  t/2667 -> concatenate20/107
  t/2668 -> concatenate20/108
  t/2669 -> concatenate20/109
  t/2670 -> concatenate20/110
  t/2671 -> concatenate20/111
  t/2672 -> concatenate20/112
  t/2673 -> concatenate20/113
  t/2674 -> concatenate20/114
  t/2675 -> concatenate20/115
  t/2676 -> concatenate20/116
  t/2677 -> concatenate20/117
  t/2678 -> concatenate20/118
  t/2679 -> concatenate20/119
  t/2680 -> concatenate20/120
  t/2681 -> concatenate20/121
  t/2682 -> concatenate20/122
  t/2683 -> concatenate20/123
  t/2684 -> concatenate20/124
  t/2685 -> concatenate20/125
  t/2686 -> concatenate20/126
  t/2687 -> concatenate20/127
  t/2688 -> concatenate20/128
  t/2689 -> concatenate21/1
  t/2690 -> concatenate21/2
  t/2691 -> concatenate21/3
  t/2692 -> concatenate21/4
  t/2693 -> concatenate21/5
  t/2694 -> concatenate21/6
  t/2695 -> concatenate21/7
  t/2696 -> concatenate21/8
  t/2697 -> concatenate21/9
  t/2698 -> concatenate21/10
  t/2699 -> concatenate21/11
  t/2700 -> concatenate21/12
  t/2701 -> concatenate21/13
  t/2702 -> concatenate21/14
  t/2703 -> concatenate21/15
  t/2704 -> concatenate21/16
  t/2705 -> concatenate21/17
  t/2706 -> concatenate21/18
  t/2707 -> concatenate21/19
  t/2708 -> concatenate21/20
  t/2709 -> concatenate21/21
  t/2710 -> concatenate21/22
  t/2711 -> concatenate21/23
  t/2712 -> concatenate21/24
  t/2713 -> concatenate21/25
  t/2714 -> concatenate21/26
  t/2715 -> concatenate21/27
  t/2716 -> concatenate21/28
  t/2717 -> concatenate21/29
  t/2718 -> concatenate21/30
  t/2719 -> concatenate21/31
  t/2720 -> concatenate21/32
  t/2721 -> concatenate21/33
  t/2722 -> concatenate21/34
  t/2723 -> concatenate21/35
  t/2724 -> concatenate21/36
  t/2725 -> concatenate21/37
  t/2726 -> concatenate21/38
  t/2727 -> concatenate21/39
  t/2728 -> concatenate21/40
  t/2729 -> concatenate21/41
  t/2730 -> concatenate21/42
  t/2731 -> concatenate21/43
  t/2732 -> concatenate21/44
  t/2733 -> concatenate21/45
  t/2734 -> concatenate21/46
  t/2735 -> concatenate21/47
  t/2736 -> concatenate21/48
  t/2737 -> concatenate21/49
  t/2738 -> concatenate21/50
  t/2739 -> concatenate21/51
  t/2740 -> concatenate21/52
  t/2741 -> concatenate21/53
  t/2742 -> concatenate21/54
  t/2743 -> concatenate21/55
  t/2744 -> concatenate21/56
  t/2745 -> concatenate21/57
  t/2746 -> concatenate21/58
  t/2747 -> concatenate21/59
  t/2748 -> concatenate21/60
  t/2749 -> concatenate21/61
  t/2750 -> concatenate21/62
  t/2751 -> concatenate21/63
  t/2752 -> concatenate21/64
  t/2753 -> concatenate21/65
  t/2754 -> concatenate21/66
  t/2755 -> concatenate21/67
  t/2756 -> concatenate21/68
  t/2757 -> concatenate21/69
  t/2758 -> concatenate21/70
  t/2759 -> concatenate21/71
  t/2760 -> concatenate21/72
  t/2761 -> concatenate21/73
  t/2762 -> concatenate21/74
  t/2763 -> concatenate21/75
  t/2764 -> concatenate21/76
  t/2765 -> concatenate21/77
  t/2766 -> concatenate21/78
  t/2767 -> concatenate21/79
  t/2768 -> concatenate21/80
  t/2769 -> concatenate21/81
  t/2770 -> concatenate21/82
  t/2771 -> concatenate21/83
  t/2772 -> concatenate21/84
  t/2773 -> concatenate21/85
  t/2774 -> concatenate21/86
  t/2775 -> concatenate21/87
  t/2776 -> concatenate21/88
  t/2777 -> concatenate21/89
  t/2778 -> concatenate21/90
  t/2779 -> concatenate21/91
  t/2780 -> concatenate21/92
  t/2781 -> concatenate21/93
  t/2782 -> concatenate21/94
  t/2783 -> concatenate21/95
  t/2784 -> concatenate21/96
  t/2785 -> concatenate21/97
  t/2786 -> concatenate21/98
  t/2787 -> concatenate21/99
  t/2788 -> concatenate21/100
  t/2789 -> concatenate21/101
  t/2790 -> concatenate21/102
  t/2791 -> concatenate21/103
  t/2792 -> concatenate21/104
  t/2793 -> concatenate21/105
  t/2794 -> concatenate21/106
  t/2795 -> concatenate21/107
  t/2796 -> concatenate21/108
  t/2797 -> concatenate21/109
  t/2798 -> concatenate21/110
  t/2799 -> concatenate21/111
  t/2800 -> concatenate21/112
  t/2801 -> concatenate21/113
  t/2802 -> concatenate21/114
  t/2803 -> concatenate21/115
  t/2804 -> concatenate21/116
  t/2805 -> concatenate21/117
  t/2806 -> concatenate21/118
  t/2807 -> concatenate21/119
  t/2808 -> concatenate21/120
  t/2809 -> concatenate21/121
  t/2810 -> concatenate21/122
  t/2811 -> concatenate21/123
  t/2812 -> concatenate21/124
  t/2813 -> concatenate21/125
  t/2814 -> concatenate21/126
  t/2815 -> concatenate21/127
  t/2816 -> concatenate21/128
  t/2817 -> concatenate22/1
  t/2818 -> concatenate22/2
  t/2819 -> concatenate22/3
  t/2820 -> concatenate22/4
  t/2821 -> concatenate22/5
  t/2822 -> concatenate22/6
  t/2823 -> concatenate22/7
  t/2824 -> concatenate22/8
  t/2825 -> concatenate22/9
  t/2826 -> concatenate22/10
  t/2827 -> concatenate22/11
  t/2828 -> concatenate22/12
  t/2829 -> concatenate22/13
  t/2830 -> concatenate22/14
  t/2831 -> concatenate22/15
  t/2832 -> concatenate22/16
  t/2833 -> concatenate22/17
  t/2834 -> concatenate22/18
  t/2835 -> concatenate22/19
  t/2836 -> concatenate22/20
  t/2837 -> concatenate22/21
  t/2838 -> concatenate22/22
  t/2839 -> concatenate22/23
  t/2840 -> concatenate22/24
  t/2841 -> concatenate22/25
  t/2842 -> concatenate22/26
  t/2843 -> concatenate22/27
  t/2844 -> concatenate22/28
  t/2845 -> concatenate22/29
  t/2846 -> concatenate22/30
  t/2847 -> concatenate22/31
  t/2848 -> concatenate22/32
  t/2849 -> concatenate22/33
  t/2850 -> concatenate22/34
  t/2851 -> concatenate22/35
  t/2852 -> concatenate22/36
  t/2853 -> concatenate22/37
  t/2854 -> concatenate22/38
  t/2855 -> concatenate22/39
  t/2856 -> concatenate22/40
  t/2857 -> concatenate22/41
  t/2858 -> concatenate22/42
  t/2859 -> concatenate22/43
  t/2860 -> concatenate22/44
  t/2861 -> concatenate22/45
  t/2862 -> concatenate22/46
  t/2863 -> concatenate22/47
  t/2864 -> concatenate22/48
  t/2865 -> concatenate22/49
  t/2866 -> concatenate22/50
  t/2867 -> concatenate22/51
  t/2868 -> concatenate22/52
  t/2869 -> concatenate22/53
  t/2870 -> concatenate22/54
  t/2871 -> concatenate22/55
  t/2872 -> concatenate22/56
  t/2873 -> concatenate22/57
  t/2874 -> concatenate22/58
  t/2875 -> concatenate22/59
  t/2876 -> concatenate22/60
  t/2877 -> concatenate22/61
  t/2878 -> concatenate22/62
  t/2879 -> concatenate22/63
  t/2880 -> concatenate22/64
  t/2881 -> concatenate22/65
  t/2882 -> concatenate22/66
  t/2883 -> concatenate22/67
  t/2884 -> concatenate22/68
  t/2885 -> concatenate22/69
  t/2886 -> concatenate22/70
  t/2887 -> concatenate22/71
  t/2888 -> concatenate22/72
  t/2889 -> concatenate22/73
  t/2890 -> concatenate22/74
  t/2891 -> concatenate22/75
  t/2892 -> concatenate22/76
  t/2893 -> concatenate22/77
  t/2894 -> concatenate22/78
  t/2895 -> concatenate22/79
  t/2896 -> concatenate22/80
  t/2897 -> concatenate22/81
  t/2898 -> concatenate22/82
  t/2899 -> concatenate22/83
  t/2900 -> concatenate22/84
  t/2901 -> concatenate22/85
  t/2902 -> concatenate22/86
  t/2903 -> concatenate22/87
  t/2904 -> concatenate22/88
  t/2905 -> concatenate22/89
  t/2906 -> concatenate22/90
  t/2907 -> concatenate22/91
  t/2908 -> concatenate22/92
  t/2909 -> concatenate22/93
  t/2910 -> concatenate22/94
  t/2911 -> concatenate22/95
  t/2912 -> concatenate22/96
  t/2913 -> concatenate22/97
  t/2914 -> concatenate22/98
  t/2915 -> concatenate22/99
  t/2916 -> concatenate22/100
  t/2917 -> concatenate22/101
  t/2918 -> concatenate22/102
  t/2919 -> concatenate22/103
  t/2920 -> concatenate22/104
  t/2921 -> concatenate22/105
  t/2922 -> concatenate22/106
  t/2923 -> concatenate22/107
  t/2924 -> concatenate22/108
  t/2925 -> concatenate22/109
  t/2926 -> concatenate22/110
  t/2927 -> concatenate22/111
  t/2928 -> concatenate22/112
  t/2929 -> concatenate22/113
  t/2930 -> concatenate22/114
  t/2931 -> concatenate22/115
  t/2932 -> concatenate22/116
  t/2933 -> concatenate22/117
  t/2934 -> concatenate22/118
  t/2935 -> concatenate22/119
  t/2936 -> concatenate22/120
  t/2937 -> concatenate22/121
  t/2938 -> concatenate22/122
  t/2939 -> concatenate22/123
  t/2940 -> concatenate22/124
  t/2941 -> concatenate22/125
  t/2942 -> concatenate22/126
  t/2943 -> concatenate22/127
  t/2944 -> concatenate22/128
  t/2945 -> concatenate23/1
  t/2946 -> concatenate23/2
  t/2947 -> concatenate23/3
  t/2948 -> concatenate23/4
  t/2949 -> concatenate23/5
  t/2950 -> concatenate23/6
  t/2951 -> concatenate23/7
  t/2952 -> concatenate23/8
  t/2953 -> concatenate23/9
  t/2954 -> concatenate23/10
  t/2955 -> concatenate23/11
  t/2956 -> concatenate23/12
  t/2957 -> concatenate23/13
  t/2958 -> concatenate23/14
  t/2959 -> concatenate23/15
  t/2960 -> concatenate23/16
  t/2961 -> concatenate23/17
  t/2962 -> concatenate23/18
  t/2963 -> concatenate23/19
  t/2964 -> concatenate23/20
  t/2965 -> concatenate23/21
  t/2966 -> concatenate23/22
  t/2967 -> concatenate23/23
  t/2968 -> concatenate23/24
  t/2969 -> concatenate23/25
  t/2970 -> concatenate23/26
  t/2971 -> concatenate23/27
  t/2972 -> concatenate23/28
  t/2973 -> concatenate23/29
  t/2974 -> concatenate23/30
  t/2975 -> concatenate23/31
  t/2976 -> concatenate23/32
  t/2977 -> concatenate23/33
  t/2978 -> concatenate23/34
  t/2979 -> concatenate23/35
  t/2980 -> concatenate23/36
  t/2981 -> concatenate23/37
  t/2982 -> concatenate23/38
  t/2983 -> concatenate23/39
  t/2984 -> concatenate23/40
  t/2985 -> concatenate23/41
  t/2986 -> concatenate23/42
  t/2987 -> concatenate23/43
  t/2988 -> concatenate23/44
  t/2989 -> concatenate23/45
  t/2990 -> concatenate23/46
  t/2991 -> concatenate23/47
  t/2992 -> concatenate23/48
  t/2993 -> concatenate23/49
  t/2994 -> concatenate23/50
  t/2995 -> concatenate23/51
  t/2996 -> concatenate23/52
  t/2997 -> concatenate23/53
  t/2998 -> concatenate23/54
  t/2999 -> concatenate23/55
  t/3000 -> concatenate23/56
  t/3001 -> concatenate23/57
  t/3002 -> concatenate23/58
  t/3003 -> concatenate23/59
  t/3004 -> concatenate23/60
  t/3005 -> concatenate23/61
  t/3006 -> concatenate23/62
  t/3007 -> concatenate23/63
  t/3008 -> concatenate23/64
  t/3009 -> concatenate23/65
  t/3010 -> concatenate23/66
  t/3011 -> concatenate23/67
  t/3012 -> concatenate23/68
  t/3013 -> concatenate23/69
  t/3014 -> concatenate23/70
  t/3015 -> concatenate23/71
  t/3016 -> concatenate23/72
  t/3017 -> concatenate23/73
  t/3018 -> concatenate23/74
  t/3019 -> concatenate23/75
  t/3020 -> concatenate23/76
  t/3021 -> concatenate23/77
  t/3022 -> concatenate23/78
  t/3023 -> concatenate23/79
  t/3024 -> concatenate23/80
  t/3025 -> concatenate23/81
  t/3026 -> concatenate23/82
  t/3027 -> concatenate23/83
  t/3028 -> concatenate23/84
  t/3029 -> concatenate23/85
  t/3030 -> concatenate23/86
  t/3031 -> concatenate23/87
  t/3032 -> concatenate23/88
  t/3033 -> concatenate23/89
  t/3034 -> concatenate23/90
  t/3035 -> concatenate23/91
  t/3036 -> concatenate23/92
  t/3037 -> concatenate23/93
  t/3038 -> concatenate23/94
  t/3039 -> concatenate23/95
  t/3040 -> concatenate23/96
  t/3041 -> concatenate23/97
  t/3042 -> concatenate23/98
  t/3043 -> concatenate23/99
  t/3044 -> concatenate23/100
  t/3045 -> concatenate23/101
  t/3046 -> concatenate23/102
  t/3047 -> concatenate23/103
  t/3048 -> concatenate23/104
  t/3049 -> concatenate23/105
  t/3050 -> concatenate23/106
  t/3051 -> concatenate23/107
  t/3052 -> concatenate23/108
  t/3053 -> concatenate23/109
  t/3054 -> concatenate23/110
  t/3055 -> concatenate23/111
  t/3056 -> concatenate23/112
  t/3057 -> concatenate23/113
  t/3058 -> concatenate23/114
  t/3059 -> concatenate23/115
  t/3060 -> concatenate23/116
  t/3061 -> concatenate23/117
  t/3062 -> concatenate23/118
  t/3063 -> concatenate23/119
  t/3064 -> concatenate23/120
  t/3065 -> concatenate23/121
  t/3066 -> concatenate23/122
  t/3067 -> concatenate23/123
  t/3068 -> concatenate23/124
  t/3069 -> concatenate23/125
  t/3070 -> concatenate23/126
  t/3071 -> concatenate23/127
  t/3072 -> concatenate23/128
  t/3073 -> concatenate24/1
  t/3074 -> concatenate24/2
  t/3075 -> concatenate24/3
  t/3076 -> concatenate24/4
  t/3077 -> concatenate24/5
  t/3078 -> concatenate24/6
  t/3079 -> concatenate24/7
  t/3080 -> concatenate24/8
  t/3081 -> concatenate24/9
  t/3082 -> concatenate24/10
  t/3083 -> concatenate24/11
  t/3084 -> concatenate24/12
  t/3085 -> concatenate24/13
  t/3086 -> concatenate24/14
  t/3087 -> concatenate24/15
  t/3088 -> concatenate24/16
  t/3089 -> concatenate24/17
  t/3090 -> concatenate24/18
  t/3091 -> concatenate24/19
  t/3092 -> concatenate24/20
  t/3093 -> concatenate24/21
  t/3094 -> concatenate24/22
  t/3095 -> concatenate24/23
  t/3096 -> concatenate24/24
  t/3097 -> concatenate24/25
  t/3098 -> concatenate24/26
  t/3099 -> concatenate24/27
  t/3100 -> concatenate24/28
  t/3101 -> concatenate24/29
  t/3102 -> concatenate24/30
  t/3103 -> concatenate24/31
  t/3104 -> concatenate24/32
  t/3105 -> concatenate24/33
  t/3106 -> concatenate24/34
  t/3107 -> concatenate24/35
  t/3108 -> concatenate24/36
  t/3109 -> concatenate24/37
  t/3110 -> concatenate24/38
  t/3111 -> concatenate24/39
  t/3112 -> concatenate24/40
  t/3113 -> concatenate24/41
  t/3114 -> concatenate24/42
  t/3115 -> concatenate24/43
  t/3116 -> concatenate24/44
  t/3117 -> concatenate24/45
  t/3118 -> concatenate24/46
  t/3119 -> concatenate24/47
  t/3120 -> concatenate24/48
  t/3121 -> concatenate24/49
  t/3122 -> concatenate24/50
  t/3123 -> concatenate24/51
  t/3124 -> concatenate24/52
  t/3125 -> concatenate24/53
  t/3126 -> concatenate24/54
  t/3127 -> concatenate24/55
  t/3128 -> concatenate24/56
  t/3129 -> concatenate24/57
  t/3130 -> concatenate24/58
  t/3131 -> concatenate24/59
  t/3132 -> concatenate24/60
  t/3133 -> concatenate24/61
  t/3134 -> concatenate24/62
  t/3135 -> concatenate24/63
  t/3136 -> concatenate24/64
  t/3137 -> concatenate24/65
  t/3138 -> concatenate24/66
  t/3139 -> concatenate24/67
  t/3140 -> concatenate24/68
  t/3141 -> concatenate24/69
  t/3142 -> concatenate24/70
  t/3143 -> concatenate24/71
  t/3144 -> concatenate24/72
  t/3145 -> concatenate24/73
  t/3146 -> concatenate24/74
  t/3147 -> concatenate24/75
  t/3148 -> concatenate24/76
  t/3149 -> concatenate24/77
  t/3150 -> concatenate24/78
  t/3151 -> concatenate24/79
  t/3152 -> concatenate24/80
  t/3153 -> concatenate24/81
  t/3154 -> concatenate24/82
  t/3155 -> concatenate24/83
  t/3156 -> concatenate24/84
  t/3157 -> concatenate24/85
  t/3158 -> concatenate24/86
  t/3159 -> concatenate24/87
  t/3160 -> concatenate24/88
  t/3161 -> concatenate24/89
  t/3162 -> concatenate24/90
  t/3163 -> concatenate24/91
  t/3164 -> concatenate24/92
  t/3165 -> concatenate24/93
  t/3166 -> concatenate24/94
  t/3167 -> concatenate24/95
  t/3168 -> concatenate24/96
  t/3169 -> concatenate24/97
  t/3170 -> concatenate24/98
  t/3171 -> concatenate24/99
  t/3172 -> concatenate24/100
  t/3173 -> concatenate24/101
  t/3174 -> concatenate24/102
  t/3175 -> concatenate24/103
  t/3176 -> concatenate24/104
  t/3177 -> concatenate24/105
  t/3178 -> concatenate24/106
  t/3179 -> concatenate24/107
  t/3180 -> concatenate24/108
  t/3181 -> concatenate24/109
  t/3182 -> concatenate24/110
  t/3183 -> concatenate24/111
  t/3184 -> concatenate24/112
  t/3185 -> concatenate24/113
  t/3186 -> concatenate24/114
  t/3187 -> concatenate24/115
  t/3188 -> concatenate24/116
  t/3189 -> concatenate24/117
  t/3190 -> concatenate24/118
  t/3191 -> concatenate24/119
  t/3192 -> concatenate24/120
  t/3193 -> concatenate24/121
  t/3194 -> concatenate24/122
  t/3195 -> concatenate24/123
  t/3196 -> concatenate24/124
  t/3197 -> concatenate24/125
  t/3198 -> concatenate24/126
  t/3199 -> concatenate24/127
  t/3200 -> concatenate24/128
  t/3201 -> concatenate25/1
  t/3202 -> concatenate25/2
  t/3203 -> concatenate25/3
  t/3204 -> concatenate25/4
  t/3205 -> concatenate25/5
  t/3206 -> concatenate25/6
  t/3207 -> concatenate25/7
  t/3208 -> concatenate25/8
  t/3209 -> concatenate25/9
  t/3210 -> concatenate25/10
  t/3211 -> concatenate25/11
  t/3212 -> concatenate25/12
  t/3213 -> concatenate25/13
  t/3214 -> concatenate25/14
  t/3215 -> concatenate25/15
  t/3216 -> concatenate25/16
  t/3217 -> concatenate25/17
  t/3218 -> concatenate25/18
  t/3219 -> concatenate25/19
  t/3220 -> concatenate25/20
  t/3221 -> concatenate25/21
  t/3222 -> concatenate25/22
  t/3223 -> concatenate25/23
  t/3224 -> concatenate25/24
  t/3225 -> concatenate25/25
  t/3226 -> concatenate25/26
  t/3227 -> concatenate25/27
  t/3228 -> concatenate25/28
  t/3229 -> concatenate25/29
  t/3230 -> concatenate25/30
  t/3231 -> concatenate25/31
  t/3232 -> concatenate25/32
  t/3233 -> concatenate25/33
  t/3234 -> concatenate25/34
  t/3235 -> concatenate25/35
  t/3236 -> concatenate25/36
  t/3237 -> concatenate25/37
  t/3238 -> concatenate25/38
  t/3239 -> concatenate25/39
  t/3240 -> concatenate25/40
  t/3241 -> concatenate25/41
  t/3242 -> concatenate25/42
  t/3243 -> concatenate25/43
  t/3244 -> concatenate25/44
  t/3245 -> concatenate25/45
  t/3246 -> concatenate25/46
  t/3247 -> concatenate25/47
  t/3248 -> concatenate25/48
  t/3249 -> concatenate25/49
  t/3250 -> concatenate25/50
  t/3251 -> concatenate25/51
  t/3252 -> concatenate25/52
  t/3253 -> concatenate25/53
  t/3254 -> concatenate25/54
  t/3255 -> concatenate25/55
  t/3256 -> concatenate25/56
  t/3257 -> concatenate25/57
  t/3258 -> concatenate25/58
  t/3259 -> concatenate25/59
  t/3260 -> concatenate25/60
  t/3261 -> concatenate25/61
  t/3262 -> concatenate25/62
  t/3263 -> concatenate25/63
  t/3264 -> concatenate25/64
  t/3265 -> concatenate25/65
  t/3266 -> concatenate25/66
  t/3267 -> concatenate25/67
  t/3268 -> concatenate25/68
  t/3269 -> concatenate25/69
  t/3270 -> concatenate25/70
  t/3271 -> concatenate25/71
  t/3272 -> concatenate25/72
  t/3273 -> concatenate25/73
  t/3274 -> concatenate25/74
  t/3275 -> concatenate25/75
  t/3276 -> concatenate25/76
  t/3277 -> concatenate25/77
  t/3278 -> concatenate25/78
  t/3279 -> concatenate25/79
  t/3280 -> concatenate25/80
  t/3281 -> concatenate25/81
  t/3282 -> concatenate25/82
  t/3283 -> concatenate25/83
  t/3284 -> concatenate25/84
  t/3285 -> concatenate25/85
  t/3286 -> concatenate25/86
  t/3287 -> concatenate25/87
  t/3288 -> concatenate25/88
  t/3289 -> concatenate25/89
  t/3290 -> concatenate25/90
  t/3291 -> concatenate25/91
  t/3292 -> concatenate25/92
  t/3293 -> concatenate25/93
  t/3294 -> concatenate25/94
  t/3295 -> concatenate25/95
  t/3296 -> concatenate25/96
  t/3297 -> concatenate25/97
  t/3298 -> concatenate25/98
  t/3299 -> concatenate25/99
  t/3300 -> concatenate25/100
  t/3301 -> concatenate25/101
  t/3302 -> concatenate25/102
  t/3303 -> concatenate25/103
  t/3304 -> concatenate25/104
  t/3305 -> concatenate25/105
  t/3306 -> concatenate25/106
  t/3307 -> concatenate25/107
  t/3308 -> concatenate25/108
  t/3309 -> concatenate25/109
  t/3310 -> concatenate25/110
  t/3311 -> concatenate25/111
  t/3312 -> concatenate25/112
  t/3313 -> concatenate25/113
  t/3314 -> concatenate25/114
  t/3315 -> concatenate25/115
  t/3316 -> concatenate25/116
  t/3317 -> concatenate25/117
  t/3318 -> concatenate25/118
  t/3319 -> concatenate25/119
  t/3320 -> concatenate25/120
  t/3321 -> concatenate25/121
  t/3322 -> concatenate25/122
  t/3323 -> concatenate25/123
  t/3324 -> concatenate25/124
  t/3325 -> concatenate25/125
  t/3326 -> concatenate25/126
  t/3327 -> concatenate25/127
  t/3328 -> concatenate25/128
  t/3329 -> concatenate26/1
  t/3330 -> concatenate26/2
  t/3331 -> concatenate26/3
  t/3332 -> concatenate26/4
  t/3333 -> concatenate26/5
  t/3334 -> concatenate26/6
  t/3335 -> concatenate26/7
  t/3336 -> concatenate26/8
  t/3337 -> concatenate26/9
  t/3338 -> concatenate26/10
  t/3339 -> concatenate26/11
  t/3340 -> concatenate26/12
  t/3341 -> concatenate26/13
  t/3342 -> concatenate26/14
  t/3343 -> concatenate26/15
  t/3344 -> concatenate26/16
  t/3345 -> concatenate26/17
  t/3346 -> concatenate26/18
  t/3347 -> concatenate26/19
  t/3348 -> concatenate26/20
  t/3349 -> concatenate26/21
  t/3350 -> concatenate26/22
  t/3351 -> concatenate26/23
  t/3352 -> concatenate26/24
  t/3353 -> concatenate26/25
  t/3354 -> concatenate26/26
  t/3355 -> concatenate26/27
  t/3356 -> concatenate26/28
  t/3357 -> concatenate26/29
  t/3358 -> concatenate26/30
  t/3359 -> concatenate26/31
  t/3360 -> concatenate26/32
  t/3361 -> concatenate26/33
  t/3362 -> concatenate26/34
  t/3363 -> concatenate26/35
  t/3364 -> concatenate26/36
  t/3365 -> concatenate26/37
  t/3366 -> concatenate26/38
  t/3367 -> concatenate26/39
  t/3368 -> concatenate26/40
  t/3369 -> concatenate26/41
  t/3370 -> concatenate26/42
  t/3371 -> concatenate26/43
  t/3372 -> concatenate26/44
  t/3373 -> concatenate26/45
  t/3374 -> concatenate26/46
  t/3375 -> concatenate26/47
  t/3376 -> concatenate26/48
  t/3377 -> concatenate26/49
  t/3378 -> concatenate26/50
  t/3379 -> concatenate26/51
  t/3380 -> concatenate26/52
  t/3381 -> concatenate26/53
  t/3382 -> concatenate26/54
  t/3383 -> concatenate26/55
  t/3384 -> concatenate26/56
  t/3385 -> concatenate26/57
  t/3386 -> concatenate26/58
  t/3387 -> concatenate26/59
  t/3388 -> concatenate26/60
  t/3389 -> concatenate26/61
  t/3390 -> concatenate26/62
  t/3391 -> concatenate26/63
  t/3392 -> concatenate26/64
  t/3393 -> concatenate26/65
  t/3394 -> concatenate26/66
  t/3395 -> concatenate26/67
  t/3396 -> concatenate26/68
  t/3397 -> concatenate26/69
  t/3398 -> concatenate26/70
  t/3399 -> concatenate26/71
  t/3400 -> concatenate26/72
  t/3401 -> concatenate26/73
  t/3402 -> concatenate26/74
  t/3403 -> concatenate26/75
  t/3404 -> concatenate26/76
  t/3405 -> concatenate26/77
  t/3406 -> concatenate26/78
  t/3407 -> concatenate26/79
  t/3408 -> concatenate26/80
  t/3409 -> concatenate26/81
  t/3410 -> concatenate26/82
  t/3411 -> concatenate26/83
  t/3412 -> concatenate26/84
  t/3413 -> concatenate26/85
  t/3414 -> concatenate26/86
  t/3415 -> concatenate26/87
  t/3416 -> concatenate26/88
  t/3417 -> concatenate26/89
  t/3418 -> concatenate26/90
  t/3419 -> concatenate26/91
  t/3420 -> concatenate26/92
  t/3421 -> concatenate26/93
  t/3422 -> concatenate26/94
  t/3423 -> concatenate26/95
  t/3424 -> concatenate26/96
  t/3425 -> concatenate26/97
  t/3426 -> concatenate26/98
  t/3427 -> concatenate26/99
  t/3428 -> concatenate26/100
  t/3429 -> concatenate26/101
  t/3430 -> concatenate26/102
  t/3431 -> concatenate26/103
  t/3432 -> concatenate26/104
  t/3433 -> concatenate26/105
  t/3434 -> concatenate26/106
  t/3435 -> concatenate26/107
  t/3436 -> concatenate26/108
  t/3437 -> concatenate26/109
  t/3438 -> concatenate26/110
  t/3439 -> concatenate26/111
  t/3440 -> concatenate26/112
  t/3441 -> concatenate26/113
  t/3442 -> concatenate26/114
  t/3443 -> concatenate26/115
  t/3444 -> concatenate26/116
  t/3445 -> concatenate26/117
  t/3446 -> concatenate26/118
  t/3447 -> concatenate26/119
  t/3448 -> concatenate26/120
  t/3449 -> concatenate26/121
  t/3450 -> concatenate26/122
  t/3451 -> concatenate26/123
  t/3452 -> concatenate26/124
  t/3453 -> concatenate26/125
  t/3454 -> concatenate26/126
  t/3455 -> concatenate26/127
  t/3456 -> concatenate26/128
  t/3457 -> concatenate27/1
  t/3458 -> concatenate27/2
  t/3459 -> concatenate27/3
  t/3460 -> concatenate27/4
  t/3461 -> concatenate27/5
  t/3462 -> concatenate27/6
  t/3463 -> concatenate27/7
  t/3464 -> concatenate27/8
  t/3465 -> concatenate27/9
  t/3466 -> concatenate27/10
  t/3467 -> concatenate27/11
  t/3468 -> concatenate27/12
  t/3469 -> concatenate27/13
  t/3470 -> concatenate27/14
  t/3471 -> concatenate27/15
  t/3472 -> concatenate27/16
  t/3473 -> concatenate27/17
  t/3474 -> concatenate27/18
  t/3475 -> concatenate27/19
  t/3476 -> concatenate27/20
  t/3477 -> concatenate27/21
  t/3478 -> concatenate27/22
  t/3479 -> concatenate27/23
  t/3480 -> concatenate27/24
  t/3481 -> concatenate27/25
  t/3482 -> concatenate27/26
  t/3483 -> concatenate27/27
  t/3484 -> concatenate27/28
  t/3485 -> concatenate27/29
  t/3486 -> concatenate27/30
  t/3487 -> concatenate27/31
  t/3488 -> concatenate27/32
  t/3489 -> concatenate27/33
  t/3490 -> concatenate27/34
  t/3491 -> concatenate27/35
  t/3492 -> concatenate27/36
  t/3493 -> concatenate27/37
  t/3494 -> concatenate27/38
  t/3495 -> concatenate27/39
  t/3496 -> concatenate27/40
  t/3497 -> concatenate27/41
  t/3498 -> concatenate27/42
  t/3499 -> concatenate27/43
  t/3500 -> concatenate27/44
  t/3501 -> concatenate27/45
  t/3502 -> concatenate27/46
  t/3503 -> concatenate27/47
  t/3504 -> concatenate27/48
  t/3505 -> concatenate27/49
  t/3506 -> concatenate27/50
  t/3507 -> concatenate27/51
  t/3508 -> concatenate27/52
  t/3509 -> concatenate27/53
  t/3510 -> concatenate27/54
  t/3511 -> concatenate27/55
  t/3512 -> concatenate27/56
  t/3513 -> concatenate27/57
  t/3514 -> concatenate27/58
  t/3515 -> concatenate27/59
  t/3516 -> concatenate27/60
  t/3517 -> concatenate27/61
  t/3518 -> concatenate27/62
  t/3519 -> concatenate27/63
  t/3520 -> concatenate27/64
  t/3521 -> concatenate27/65
  t/3522 -> concatenate27/66
  t/3523 -> concatenate27/67
  t/3524 -> concatenate27/68
  t/3525 -> concatenate27/69
  t/3526 -> concatenate27/70
  t/3527 -> concatenate27/71
  t/3528 -> concatenate27/72
  t/3529 -> concatenate27/73
  t/3530 -> concatenate27/74
  t/3531 -> concatenate27/75
  t/3532 -> concatenate27/76
  t/3533 -> concatenate27/77
  t/3534 -> concatenate27/78
  t/3535 -> concatenate27/79
  t/3536 -> concatenate27/80
  t/3537 -> concatenate27/81
  t/3538 -> concatenate27/82
  t/3539 -> concatenate27/83
  t/3540 -> concatenate27/84
  t/3541 -> concatenate27/85
  t/3542 -> concatenate27/86
  t/3543 -> concatenate27/87
  t/3544 -> concatenate27/88
  t/3545 -> concatenate27/89
  t/3546 -> concatenate27/90
  t/3547 -> concatenate27/91
  t/3548 -> concatenate27/92
  t/3549 -> concatenate27/93
  t/3550 -> concatenate27/94
  t/3551 -> concatenate27/95
  t/3552 -> concatenate27/96
  t/3553 -> concatenate27/97
  t/3554 -> concatenate27/98
  t/3555 -> concatenate27/99
  t/3556 -> concatenate27/100
  t/3557 -> concatenate27/101
  t/3558 -> concatenate27/102
  t/3559 -> concatenate27/103
  t/3560 -> concatenate27/104
  t/3561 -> concatenate27/105
  t/3562 -> concatenate27/106
  t/3563 -> concatenate27/107
  t/3564 -> concatenate27/108
  t/3565 -> concatenate27/109
  t/3566 -> concatenate27/110
  t/3567 -> concatenate27/111
  t/3568 -> concatenate27/112
  t/3569 -> concatenate27/113
  t/3570 -> concatenate27/114
  t/3571 -> concatenate27/115
  t/3572 -> concatenate27/116
  t/3573 -> concatenate27/117
  t/3574 -> concatenate27/118
  t/3575 -> concatenate27/119
  t/3576 -> concatenate27/120
  t/3577 -> concatenate27/121
  t/3578 -> concatenate27/122
  t/3579 -> concatenate27/123
  t/3580 -> concatenate27/124
  t/3581 -> concatenate27/125
  t/3582 -> concatenate27/126
  t/3583 -> concatenate27/127
  t/3584 -> concatenate27/128
  t/3585 -> concatenate28/1
  t/3586 -> concatenate28/2
  t/3587 -> concatenate28/3
  t/3588 -> concatenate28/4
  t/3589 -> concatenate28/5
  t/3590 -> concatenate28/6
  t/3591 -> concatenate28/7
  t/3592 -> concatenate28/8
  t/3593 -> concatenate28/9
  t/3594 -> concatenate28/10
  t/3595 -> concatenate28/11
  t/3596 -> concatenate28/12
  t/3597 -> concatenate28/13
  t/3598 -> concatenate28/14
  t/3599 -> concatenate28/15
  t/3600 -> concatenate28/16
  t/3601 -> concatenate28/17
  t/3602 -> concatenate28/18
  t/3603 -> concatenate28/19
  t/3604 -> concatenate28/20
  t/3605 -> concatenate28/21
  t/3606 -> concatenate28/22
  t/3607 -> concatenate28/23
  t/3608 -> concatenate28/24
  t/3609 -> concatenate28/25
  t/3610 -> concatenate28/26
  t/3611 -> concatenate28/27
  t/3612 -> concatenate28/28
  t/3613 -> concatenate28/29
  t/3614 -> concatenate28/30
  t/3615 -> concatenate28/31
  t/3616 -> concatenate28/32
  t/3617 -> concatenate28/33
  t/3618 -> concatenate28/34
  t/3619 -> concatenate28/35
  t/3620 -> concatenate28/36
  t/3621 -> concatenate28/37
  t/3622 -> concatenate28/38
  t/3623 -> concatenate28/39
  t/3624 -> concatenate28/40
  t/3625 -> concatenate28/41
  t/3626 -> concatenate28/42
  t/3627 -> concatenate28/43
  t/3628 -> concatenate28/44
  t/3629 -> concatenate28/45
  t/3630 -> concatenate28/46
  t/3631 -> concatenate28/47
  t/3632 -> concatenate28/48
  t/3633 -> concatenate28/49
  t/3634 -> concatenate28/50
  t/3635 -> concatenate28/51
  t/3636 -> concatenate28/52
  t/3637 -> concatenate28/53
  t/3638 -> concatenate28/54
  t/3639 -> concatenate28/55
  t/3640 -> concatenate28/56
  t/3641 -> concatenate28/57
  t/3642 -> concatenate28/58
  t/3643 -> concatenate28/59
  t/3644 -> concatenate28/60
  t/3645 -> concatenate28/61
  t/3646 -> concatenate28/62
  t/3647 -> concatenate28/63
  t/3648 -> concatenate28/64
  t/3649 -> concatenate28/65
  t/3650 -> concatenate28/66
  t/3651 -> concatenate28/67
  t/3652 -> concatenate28/68
  t/3653 -> concatenate28/69
  t/3654 -> concatenate28/70
  t/3655 -> concatenate28/71
  t/3656 -> concatenate28/72
  t/3657 -> concatenate28/73
  t/3658 -> concatenate28/74
  t/3659 -> concatenate28/75
  t/3660 -> concatenate28/76
  t/3661 -> concatenate28/77
  t/3662 -> concatenate28/78
  t/3663 -> concatenate28/79
  t/3664 -> concatenate28/80
  t/3665 -> concatenate28/81
  t/3666 -> concatenate28/82
  t/3667 -> concatenate28/83
  t/3668 -> concatenate28/84
  t/3669 -> concatenate28/85
  t/3670 -> concatenate28/86
  t/3671 -> concatenate28/87
  t/3672 -> concatenate28/88
  t/3673 -> concatenate28/89
  t/3674 -> concatenate28/90
  t/3675 -> concatenate28/91
  t/3676 -> concatenate28/92
  t/3677 -> concatenate28/93
  t/3678 -> concatenate28/94
  t/3679 -> concatenate28/95
  t/3680 -> concatenate28/96
  t/3681 -> concatenate28/97
  t/3682 -> concatenate28/98
  t/3683 -> concatenate28/99
  t/3684 -> concatenate28/100
  t/3685 -> concatenate28/101
  t/3686 -> concatenate28/102
  t/3687 -> concatenate28/103
  t/3688 -> concatenate28/104
  t/3689 -> concatenate28/105
  t/3690 -> concatenate28/106
  t/3691 -> concatenate28/107
  t/3692 -> concatenate28/108
  t/3693 -> concatenate28/109
  t/3694 -> concatenate28/110
  t/3695 -> concatenate28/111
  t/3696 -> concatenate28/112
  t/3697 -> concatenate28/113
  t/3698 -> concatenate28/114
  t/3699 -> concatenate28/115
  t/3700 -> concatenate28/116
  t/3701 -> concatenate28/117
  t/3702 -> concatenate28/118
  t/3703 -> concatenate28/119
  t/3704 -> concatenate28/120
  t/3705 -> concatenate28/121
  t/3706 -> concatenate28/122
  t/3707 -> concatenate28/123
  t/3708 -> concatenate28/124
  t/3709 -> concatenate28/125
  t/3710 -> concatenate28/126
  t/3711 -> concatenate28/127
  t/3712 -> concatenate28/128
  t/3713 -> concatenate29/1
  t/3714 -> concatenate29/2
  t/3715 -> concatenate29/3
  t/3716 -> concatenate29/4
  t/3717 -> concatenate29/5
  t/3718 -> concatenate29/6
  t/3719 -> concatenate29/7
  t/3720 -> concatenate29/8
  t/3721 -> concatenate29/9
  t/3722 -> concatenate29/10
  t/3723 -> concatenate29/11
  t/3724 -> concatenate29/12
  t/3725 -> concatenate29/13
  t/3726 -> concatenate29/14
  t/3727 -> concatenate29/15
  t/3728 -> concatenate29/16
  t/3729 -> concatenate29/17
  t/3730 -> concatenate29/18
  t/3731 -> concatenate29/19
  t/3732 -> concatenate29/20
  t/3733 -> concatenate29/21
  t/3734 -> concatenate29/22
  t/3735 -> concatenate29/23
  t/3736 -> concatenate29/24
  t/3737 -> concatenate29/25
  t/3738 -> concatenate29/26
  t/3739 -> concatenate29/27
  t/3740 -> concatenate29/28
  t/3741 -> concatenate29/29
  t/3742 -> concatenate29/30
  t/3743 -> concatenate29/31
  t/3744 -> concatenate29/32
  t/3745 -> concatenate29/33
  t/3746 -> concatenate29/34
  t/3747 -> concatenate29/35
  t/3748 -> concatenate29/36
  t/3749 -> concatenate29/37
  t/3750 -> concatenate29/38
  t/3751 -> concatenate29/39
  t/3752 -> concatenate29/40
  t/3753 -> concatenate29/41
  t/3754 -> concatenate29/42
  t/3755 -> concatenate29/43
  t/3756 -> concatenate29/44
  t/3757 -> concatenate29/45
  t/3758 -> concatenate29/46
  t/3759 -> concatenate29/47
  t/3760 -> concatenate29/48
  t/3761 -> concatenate29/49
  t/3762 -> concatenate29/50
  t/3763 -> concatenate29/51
  t/3764 -> concatenate29/52
  t/3765 -> concatenate29/53
  t/3766 -> concatenate29/54
  t/3767 -> concatenate29/55
  t/3768 -> concatenate29/56
  t/3769 -> concatenate29/57
  t/3770 -> concatenate29/58
  t/3771 -> concatenate29/59
  t/3772 -> concatenate29/60
  t/3773 -> concatenate29/61
  t/3774 -> concatenate29/62
  t/3775 -> concatenate29/63
  t/3776 -> concatenate29/64
  t/3777 -> concatenate29/65
  t/3778 -> concatenate29/66
  t/3779 -> concatenate29/67
  t/3780 -> concatenate29/68
  t/3781 -> concatenate29/69
  t/3782 -> concatenate29/70
  t/3783 -> concatenate29/71
  t/3784 -> concatenate29/72
  t/3785 -> concatenate29/73
  t/3786 -> concatenate29/74
  t/3787 -> concatenate29/75
  t/3788 -> concatenate29/76
  t/3789 -> concatenate29/77
  t/3790 -> concatenate29/78
  t/3791 -> concatenate29/79
  t/3792 -> concatenate29/80
  t/3793 -> concatenate29/81
  t/3794 -> concatenate29/82
  t/3795 -> concatenate29/83
  t/3796 -> concatenate29/84
  t/3797 -> concatenate29/85
  t/3798 -> concatenate29/86
  t/3799 -> concatenate29/87
  t/3800 -> concatenate29/88
  t/3801 -> concatenate29/89
  t/3802 -> concatenate29/90
  t/3803 -> concatenate29/91
  t/3804 -> concatenate29/92
  t/3805 -> concatenate29/93
  t/3806 -> concatenate29/94
  t/3807 -> concatenate29/95
  t/3808 -> concatenate29/96
  t/3809 -> concatenate29/97
  t/3810 -> concatenate29/98
  t/3811 -> concatenate29/99
  t/3812 -> concatenate29/100
  t/3813 -> concatenate29/101
  t/3814 -> concatenate29/102
  t/3815 -> concatenate29/103
  t/3816 -> concatenate29/104
  t/3817 -> concatenate29/105
  t/3818 -> concatenate29/106
  t/3819 -> concatenate29/107
  t/3820 -> concatenate29/108
  t/3821 -> concatenate29/109
  t/3822 -> concatenate29/110
  t/3823 -> concatenate29/111
  t/3824 -> concatenate29/112
  t/3825 -> concatenate29/113
  t/3826 -> concatenate29/114
  t/3827 -> concatenate29/115
  t/3828 -> concatenate29/116
  t/3829 -> concatenate29/117
  t/3830 -> concatenate29/118
  t/3831 -> concatenate29/119
  t/3832 -> concatenate29/120
  t/3833 -> concatenate29/121
  t/3834 -> concatenate29/122
  t/3835 -> concatenate29/123
  t/3836 -> concatenate29/124
  t/3837 -> concatenate29/125
  t/3838 -> concatenate29/126
  t/3839 -> concatenate29/127
  t/3840 -> concatenate29/128
  t/3841 -> concatenate30/1
  t/3842 -> concatenate30/2
  t/3843 -> concatenate30/3
  t/3844 -> concatenate30/4
  t/3845 -> concatenate30/5
  t/3846 -> concatenate30/6
  t/3847 -> concatenate30/7
  t/3848 -> concatenate30/8
  t/3849 -> concatenate30/9
  t/3850 -> concatenate30/10
  t/3851 -> concatenate30/11
  t/3852 -> concatenate30/12
  t/3853 -> concatenate30/13
  t/3854 -> concatenate30/14
  t/3855 -> concatenate30/15
  t/3856 -> concatenate30/16
  t/3857 -> concatenate30/17
  t/3858 -> concatenate30/18
  t/3859 -> concatenate30/19
  t/3860 -> concatenate30/20
  t/3861 -> concatenate30/21
  t/3862 -> concatenate30/22
  t/3863 -> concatenate30/23
  t/3864 -> concatenate30/24
  t/3865 -> concatenate30/25
  t/3866 -> concatenate30/26
  t/3867 -> concatenate30/27
  t/3868 -> concatenate30/28
  t/3869 -> concatenate30/29
  t/3870 -> concatenate30/30
  t/3871 -> concatenate30/31
  t/3872 -> concatenate30/32
  t/3873 -> concatenate30/33
  t/3874 -> concatenate30/34
  t/3875 -> concatenate30/35
  t/3876 -> concatenate30/36
  t/3877 -> concatenate30/37
  t/3878 -> concatenate30/38
  t/3879 -> concatenate30/39
  t/3880 -> concatenate30/40
  t/3881 -> concatenate30/41
  t/3882 -> concatenate30/42
  t/3883 -> concatenate30/43
  t/3884 -> concatenate30/44
  t/3885 -> concatenate30/45
  t/3886 -> concatenate30/46
  t/3887 -> concatenate30/47
  t/3888 -> concatenate30/48
  t/3889 -> concatenate30/49
  t/3890 -> concatenate30/50
  t/3891 -> concatenate30/51
  t/3892 -> concatenate30/52
  t/3893 -> concatenate30/53
  t/3894 -> concatenate30/54
  t/3895 -> concatenate30/55
  t/3896 -> concatenate30/56
  t/3897 -> concatenate30/57
  t/3898 -> concatenate30/58
  t/3899 -> concatenate30/59
  t/3900 -> concatenate30/60
  t/3901 -> concatenate30/61
  t/3902 -> concatenate30/62
  t/3903 -> concatenate30/63
  t/3904 -> concatenate30/64
  t/3905 -> concatenate30/65
  t/3906 -> concatenate30/66
  t/3907 -> concatenate30/67
  t/3908 -> concatenate30/68
  t/3909 -> concatenate30/69
  t/3910 -> concatenate30/70
  t/3911 -> concatenate30/71
  t/3912 -> concatenate30/72
  t/3913 -> concatenate30/73
  t/3914 -> concatenate30/74
  t/3915 -> concatenate30/75
  t/3916 -> concatenate30/76
  t/3917 -> concatenate30/77
  t/3918 -> concatenate30/78
  t/3919 -> concatenate30/79
  t/3920 -> concatenate30/80
  t/3921 -> concatenate30/81
  t/3922 -> concatenate30/82
  t/3923 -> concatenate30/83
  t/3924 -> concatenate30/84
  t/3925 -> concatenate30/85
  t/3926 -> concatenate30/86
  t/3927 -> concatenate30/87
  t/3928 -> concatenate30/88
  t/3929 -> concatenate30/89
  t/3930 -> concatenate30/90
  t/3931 -> concatenate30/91
  t/3932 -> concatenate30/92
  t/3933 -> concatenate30/93
  t/3934 -> concatenate30/94
  t/3935 -> concatenate30/95
  t/3936 -> concatenate30/96
  t/3937 -> concatenate30/97
  t/3938 -> concatenate30/98
  t/3939 -> concatenate30/99
  t/3940 -> concatenate30/100
  t/3941 -> concatenate30/101
  t/3942 -> concatenate30/102
  t/3943 -> concatenate30/103
  t/3944 -> concatenate30/104
  t/3945 -> concatenate30/105
  t/3946 -> concatenate30/106
  t/3947 -> concatenate30/107
  t/3948 -> concatenate30/108
  t/3949 -> concatenate30/109
  t/3950 -> concatenate30/110
  t/3951 -> concatenate30/111
  t/3952 -> concatenate30/112
  t/3953 -> concatenate30/113
  t/3954 -> concatenate30/114
  t/3955 -> concatenate30/115
  t/3956 -> concatenate30/116
  t/3957 -> concatenate30/117
  t/3958 -> concatenate30/118
  t/3959 -> concatenate30/119
  t/3960 -> concatenate30/120
  t/3961 -> concatenate30/121
  t/3962 -> concatenate30/122
  t/3963 -> concatenate30/123
  t/3964 -> concatenate30/124
  t/3965 -> concatenate30/125
  t/3966 -> concatenate30/126
  t/3967 -> concatenate30/127
  t/3968 -> concatenate30/128
  t/3969 -> concatenate31/1
  t/3970 -> concatenate31/2
  t/3971 -> concatenate31/3
  t/3972 -> concatenate31/4
  t/3973 -> concatenate31/5
  t/3974 -> concatenate31/6
  t/3975 -> concatenate31/7
  t/3976 -> concatenate31/8
  t/3977 -> concatenate31/9
  t/3978 -> concatenate31/10
  t/3979 -> concatenate31/11
  t/3980 -> concatenate31/12
  t/3981 -> concatenate31/13
  t/3982 -> concatenate31/14
  t/3983 -> concatenate31/15
  t/3984 -> concatenate31/16
  t/3985 -> concatenate31/17
  t/3986 -> concatenate31/18
  t/3987 -> concatenate31/19
  t/3988 -> concatenate31/20
  t/3989 -> concatenate31/21
  t/3990 -> concatenate31/22
  t/3991 -> concatenate31/23
  t/3992 -> concatenate31/24
  t/3993 -> concatenate31/25
  t/3994 -> concatenate31/26
  t/3995 -> concatenate31/27
  t/3996 -> concatenate31/28
  t/3997 -> concatenate31/29
  t/3998 -> concatenate31/30
  t/3999 -> concatenate31/31
  t/4000 -> concatenate31/32
  t/4001 -> concatenate31/33
  t/4002 -> concatenate31/34
  t/4003 -> concatenate31/35
  t/4004 -> concatenate31/36
  t/4005 -> concatenate31/37
  t/4006 -> concatenate31/38
  t/4007 -> concatenate31/39
  t/4008 -> concatenate31/40
  t/4009 -> concatenate31/41
  t/4010 -> concatenate31/42
  t/4011 -> concatenate31/43
  t/4012 -> concatenate31/44
  t/4013 -> concatenate31/45
  t/4014 -> concatenate31/46
  t/4015 -> concatenate31/47
  t/4016 -> concatenate31/48
  t/4017 -> concatenate31/49
  t/4018 -> concatenate31/50
  t/4019 -> concatenate31/51
  t/4020 -> concatenate31/52
  t/4021 -> concatenate31/53
  t/4022 -> concatenate31/54
  t/4023 -> concatenate31/55
  t/4024 -> concatenate31/56
  t/4025 -> concatenate31/57
  t/4026 -> concatenate31/58
  t/4027 -> concatenate31/59
  t/4028 -> concatenate31/60
  t/4029 -> concatenate31/61
  t/4030 -> concatenate31/62
  t/4031 -> concatenate31/63
  t/4032 -> concatenate31/64
  t/4033 -> concatenate31/65
  t/4034 -> concatenate31/66
  t/4035 -> concatenate31/67
  t/4036 -> concatenate31/68
  t/4037 -> concatenate31/69
  t/4038 -> concatenate31/70
  t/4039 -> concatenate31/71
  t/4040 -> concatenate31/72
  t/4041 -> concatenate31/73
  t/4042 -> concatenate31/74
  t/4043 -> concatenate31/75
  t/4044 -> concatenate31/76
  t/4045 -> concatenate31/77
  t/4046 -> concatenate31/78
  t/4047 -> concatenate31/79
  t/4048 -> concatenate31/80
  t/4049 -> concatenate31/81
  t/4050 -> concatenate31/82
  t/4051 -> concatenate31/83
  t/4052 -> concatenate31/84
  t/4053 -> concatenate31/85
  t/4054 -> concatenate31/86
  t/4055 -> concatenate31/87
  t/4056 -> concatenate31/88
  t/4057 -> concatenate31/89
  t/4058 -> concatenate31/90
  t/4059 -> concatenate31/91
  t/4060 -> concatenate31/92
  t/4061 -> concatenate31/93
  t/4062 -> concatenate31/94
  t/4063 -> concatenate31/95
  t/4064 -> concatenate31/96
  t/4065 -> concatenate31/97
  t/4066 -> concatenate31/98
  t/4067 -> concatenate31/99
  t/4068 -> concatenate31/100
  t/4069 -> concatenate31/101
  t/4070 -> concatenate31/102
  t/4071 -> concatenate31/103
  t/4072 -> concatenate31/104
  t/4073 -> concatenate31/105
  t/4074 -> concatenate31/106
  t/4075 -> concatenate31/107
  t/4076 -> concatenate31/108
  t/4077 -> concatenate31/109
  t/4078 -> concatenate31/110
  t/4079 -> concatenate31/111
  t/4080 -> concatenate31/112
  t/4081 -> concatenate31/113
  t/4082 -> concatenate31/114
  t/4083 -> concatenate31/115
  t/4084 -> concatenate31/116
  t/4085 -> concatenate31/117
  t/4086 -> concatenate31/118
  t/4087 -> concatenate31/119
  t/4088 -> concatenate31/120
  t/4089 -> concatenate31/121
  t/4090 -> concatenate31/122
  t/4091 -> concatenate31/123
  t/4092 -> concatenate31/124
  t/4093 -> concatenate31/125
  t/4094 -> concatenate31/126
  t/4095 -> concatenate31/127
  t/4096 -> concatenate31/128
  t/4097 -> concatenate32/1
  t/4098 -> concatenate32/2
  t/4099 -> concatenate32/3
  t/4100 -> concatenate32/4
  t/4101 -> concatenate32/5
  t/4102 -> concatenate32/6
  t/4103 -> concatenate32/7
  t/4104 -> concatenate32/8
  t/4105 -> concatenate32/9
  t/4106 -> concatenate32/10
  t/4107 -> concatenate32/11
  t/4108 -> concatenate32/12
  t/4109 -> concatenate32/13
  t/4110 -> concatenate32/14
  t/4111 -> concatenate32/15
  t/4112 -> concatenate32/16
  t/4113 -> concatenate32/17
  t/4114 -> concatenate32/18
  t/4115 -> concatenate32/19
  t/4116 -> concatenate32/20
  t/4117 -> concatenate32/21
  t/4118 -> concatenate32/22
  t/4119 -> concatenate32/23
  t/4120 -> concatenate32/24
  t/4121 -> concatenate32/25
  t/4122 -> concatenate32/26
  t/4123 -> concatenate32/27
  t/4124 -> concatenate32/28
  t/4125 -> concatenate32/29
  t/4126 -> concatenate32/30
  t/4127 -> concatenate32/31
  t/4128 -> concatenate32/32
  t/4129 -> concatenate32/33
  t/4130 -> concatenate32/34
  t/4131 -> concatenate32/35
  t/4132 -> concatenate32/36
  t/4133 -> concatenate32/37
  t/4134 -> concatenate32/38
  t/4135 -> concatenate32/39
  t/4136 -> concatenate32/40
  t/4137 -> concatenate32/41
  t/4138 -> concatenate32/42
  t/4139 -> concatenate32/43
  t/4140 -> concatenate32/44
  t/4141 -> concatenate32/45
  t/4142 -> concatenate32/46
  t/4143 -> concatenate32/47
  t/4144 -> concatenate32/48
  t/4145 -> concatenate32/49
  t/4146 -> concatenate32/50
  t/4147 -> concatenate32/51
  t/4148 -> concatenate32/52
  t/4149 -> concatenate32/53
  t/4150 -> concatenate32/54
  t/4151 -> concatenate32/55
  t/4152 -> concatenate32/56
  t/4153 -> concatenate32/57
  t/4154 -> concatenate32/58
  t/4155 -> concatenate32/59
  t/4156 -> concatenate32/60
  t/4157 -> concatenate32/61
  t/4158 -> concatenate32/62
  t/4159 -> concatenate32/63
  t/4160 -> concatenate32/64
  t/4161 -> concatenate32/65
  t/4162 -> concatenate32/66
  t/4163 -> concatenate32/67
  t/4164 -> concatenate32/68
  t/4165 -> concatenate32/69
  t/4166 -> concatenate32/70
  t/4167 -> concatenate32/71
  t/4168 -> concatenate32/72
  t/4169 -> concatenate32/73
  t/4170 -> concatenate32/74
  t/4171 -> concatenate32/75
  t/4172 -> concatenate32/76
  t/4173 -> concatenate32/77
  t/4174 -> concatenate32/78
  t/4175 -> concatenate32/79
  t/4176 -> concatenate32/80
  t/4177 -> concatenate32/81
  t/4178 -> concatenate32/82
  t/4179 -> concatenate32/83
  t/4180 -> concatenate32/84
  t/4181 -> concatenate32/85
  t/4182 -> concatenate32/86
  t/4183 -> concatenate32/87
  t/4184 -> concatenate32/88
  t/4185 -> concatenate32/89
  t/4186 -> concatenate32/90
  t/4187 -> concatenate32/91
  t/4188 -> concatenate32/92
  t/4189 -> concatenate32/93
  t/4190 -> concatenate32/94
  t/4191 -> concatenate32/95
  t/4192 -> concatenate32/96
  t/4193 -> concatenate32/97
  t/4194 -> concatenate32/98
  t/4195 -> concatenate32/99
  t/4196 -> concatenate32/100
  t/4197 -> concatenate32/101
  t/4198 -> concatenate32/102
  t/4199 -> concatenate32/103
  t/4200 -> concatenate32/104
  t/4201 -> concatenate32/105
  t/4202 -> concatenate32/106
  t/4203 -> concatenate32/107
  t/4204 -> concatenate32/108
  t/4205 -> concatenate32/109
  t/4206 -> concatenate32/110
  t/4207 -> concatenate32/111
  t/4208 -> concatenate32/112
  t/4209 -> concatenate32/113
  t/4210 -> concatenate32/114
  t/4211 -> concatenate32/115
  t/4212 -> concatenate32/116
  t/4213 -> concatenate32/117
  t/4214 -> concatenate32/118
  t/4215 -> concatenate32/119
  t/4216 -> concatenate32/120
  t/4217 -> concatenate32/121
  t/4218 -> concatenate32/122
  t/4219 -> concatenate32/123
  t/4220 -> concatenate32/124
  t/4221 -> concatenate32/125
  t/4222 -> concatenate32/126
  t/4223 -> concatenate32/127
  t/4224 -> concatenate32/128
  t/4225 -> concatenate33/1
  t/4226 -> concatenate33/2
  t/4227 -> concatenate33/3
  t/4228 -> concatenate33/4
  t/4229 -> concatenate33/5
  t/4230 -> concatenate33/6
  t/4231 -> concatenate33/7
  t/4232 -> concatenate33/8
  t/4233 -> concatenate33/9
  t/4234 -> concatenate33/10
  t/4235 -> concatenate33/11
  t/4236 -> concatenate33/12
  t/4237 -> concatenate33/13
  t/4238 -> concatenate33/14
  t/4239 -> concatenate33/15
  t/4240 -> concatenate33/16
  t/4241 -> concatenate33/17
  t/4242 -> concatenate33/18
  t/4243 -> concatenate33/19
  t/4244 -> concatenate33/20
  t/4245 -> concatenate33/21
  t/4246 -> concatenate33/22
  t/4247 -> concatenate33/23
  t/4248 -> concatenate33/24
  t/4249 -> concatenate33/25
  t/4250 -> concatenate33/26
  t/4251 -> concatenate33/27
  t/4252 -> concatenate33/28
  t/4253 -> concatenate33/29
  t/4254 -> concatenate33/30
  t/4255 -> concatenate33/31
  t/4256 -> concatenate33/32
  t/4257 -> concatenate33/33
  t/4258 -> concatenate33/34
  t/4259 -> concatenate33/35
  t/4260 -> concatenate33/36
  t/4261 -> concatenate33/37
  t/4262 -> concatenate33/38
  t/4263 -> concatenate33/39
  t/4264 -> concatenate33/40
  t/4265 -> concatenate33/41
  t/4266 -> concatenate33/42
  t/4267 -> concatenate33/43
  t/4268 -> concatenate33/44
  t/4269 -> concatenate33/45
  t/4270 -> concatenate33/46
  t/4271 -> concatenate33/47
  t/4272 -> concatenate33/48
  t/4273 -> concatenate33/49
  t/4274 -> concatenate33/50
  t/4275 -> concatenate33/51
  t/4276 -> concatenate33/52
  t/4277 -> concatenate33/53
  t/4278 -> concatenate33/54
  t/4279 -> concatenate33/55
  t/4280 -> concatenate33/56
  t/4281 -> concatenate33/57
  t/4282 -> concatenate33/58
  t/4283 -> concatenate33/59
  t/4284 -> concatenate33/60
  t/4285 -> concatenate33/61
  t/4286 -> concatenate33/62
  t/4287 -> concatenate33/63
  t/4288 -> concatenate33/64
  t/4289 -> concatenate33/65
  t/4290 -> concatenate33/66
  t/4291 -> concatenate33/67
  t/4292 -> concatenate33/68
  t/4293 -> concatenate33/69
  t/4294 -> concatenate33/70
  t/4295 -> concatenate33/71
  t/4296 -> concatenate33/72
  t/4297 -> concatenate33/73
  t/4298 -> concatenate33/74
  t/4299 -> concatenate33/75
  t/4300 -> concatenate33/76
  t/4301 -> concatenate33/77
  t/4302 -> concatenate33/78
  t/4303 -> concatenate33/79
  t/4304 -> concatenate33/80
  t/4305 -> concatenate33/81
  t/4306 -> concatenate33/82
  t/4307 -> concatenate33/83
  t/4308 -> concatenate33/84
  t/4309 -> concatenate33/85
  t/4310 -> concatenate33/86
  t/4311 -> concatenate33/87
  t/4312 -> concatenate33/88
  t/4313 -> concatenate33/89
  t/4314 -> concatenate33/90
  t/4315 -> concatenate33/91
  t/4316 -> concatenate33/92
  t/4317 -> concatenate33/93
  t/4318 -> concatenate33/94
  t/4319 -> concatenate33/95
  t/4320 -> concatenate33/96
  t/4321 -> concatenate33/97
  t/4322 -> concatenate33/98
  t/4323 -> concatenate33/99
  t/4324 -> concatenate33/100
  t/4325 -> concatenate33/101
  t/4326 -> concatenate33/102
  t/4327 -> concatenate33/103
  t/4328 -> concatenate33/104
  t/4329 -> concatenate33/105
  t/4330 -> concatenate33/106
  t/4331 -> concatenate33/107
  t/4332 -> concatenate33/108
  t/4333 -> concatenate33/109
  t/4334 -> concatenate33/110
  t/4335 -> concatenate33/111
  t/4336 -> concatenate33/112
  t/4337 -> concatenate33/113
  t/4338 -> concatenate33/114
  t/4339 -> concatenate33/115
  t/4340 -> concatenate33/116
  t/4341 -> concatenate33/117
  t/4342 -> concatenate33/118
  t/4343 -> concatenate33/119
  t/4344 -> concatenate33/120
  t/4345 -> concatenate33/121
  t/4346 -> concatenate33/122
  t/4347 -> concatenate33/123
  t/4348 -> concatenate33/124
  t/4349 -> concatenate33/125
  t/4350 -> concatenate33/126
  t/4351 -> concatenate33/127
  t/4352 -> concatenate33/128
  t/4353 -> concatenate34/1
  t/4354 -> concatenate34/2
  t/4355 -> concatenate34/3
  t/4356 -> concatenate34/4
  t/4357 -> concatenate34/5
  t/4358 -> concatenate34/6
  t/4359 -> concatenate34/7
  t/4360 -> concatenate34/8
  t/4361 -> concatenate34/9
  t/4362 -> concatenate34/10
  t/4363 -> concatenate34/11
  t/4364 -> concatenate34/12
  t/4365 -> concatenate34/13
  t/4366 -> concatenate34/14
  t/4367 -> concatenate34/15
  t/4368 -> concatenate34/16
  t/4369 -> concatenate34/17
  t/4370 -> concatenate34/18
  t/4371 -> concatenate34/19
  t/4372 -> concatenate34/20
  t/4373 -> concatenate34/21
  t/4374 -> concatenate34/22
  t/4375 -> concatenate34/23
  t/4376 -> concatenate34/24
  t/4377 -> concatenate34/25
  t/4378 -> concatenate34/26
  t/4379 -> concatenate34/27
  t/4380 -> concatenate34/28
  t/4381 -> concatenate34/29
  t/4382 -> concatenate34/30
  t/4383 -> concatenate34/31
  t/4384 -> concatenate34/32
  t/4385 -> concatenate34/33
  t/4386 -> concatenate34/34
  t/4387 -> concatenate34/35
  t/4388 -> concatenate34/36
  t/4389 -> concatenate34/37
  t/4390 -> concatenate34/38
  t/4391 -> concatenate34/39
  t/4392 -> concatenate34/40
  t/4393 -> concatenate34/41
  t/4394 -> concatenate34/42
  t/4395 -> concatenate34/43
  t/4396 -> concatenate34/44
  t/4397 -> concatenate34/45
  t/4398 -> concatenate34/46
  t/4399 -> concatenate34/47
  t/4400 -> concatenate34/48
  t/4401 -> concatenate34/49
  t/4402 -> concatenate34/50
  t/4403 -> concatenate34/51
  t/4404 -> concatenate34/52
  t/4405 -> concatenate34/53
  t/4406 -> concatenate34/54
  t/4407 -> concatenate34/55
  t/4408 -> concatenate34/56
  t/4409 -> concatenate34/57
  t/4410 -> concatenate34/58
  t/4411 -> concatenate34/59
  t/4412 -> concatenate34/60
  t/4413 -> concatenate34/61
  t/4414 -> concatenate34/62
  t/4415 -> concatenate34/63
  t/4416 -> concatenate34/64
  t/4417 -> concatenate34/65
  t/4418 -> concatenate34/66
  t/4419 -> concatenate34/67
  t/4420 -> concatenate34/68
  t/4421 -> concatenate34/69
  t/4422 -> concatenate34/70
  t/4423 -> concatenate34/71
  t/4424 -> concatenate34/72
  t/4425 -> concatenate34/73
  t/4426 -> concatenate34/74
  t/4427 -> concatenate34/75
  t/4428 -> concatenate34/76
  t/4429 -> concatenate34/77
  t/4430 -> concatenate34/78
  t/4431 -> concatenate34/79
  t/4432 -> concatenate34/80
  t/4433 -> concatenate34/81
  t/4434 -> concatenate34/82
  t/4435 -> concatenate34/83
  t/4436 -> concatenate34/84
  t/4437 -> concatenate34/85
  t/4438 -> concatenate34/86
  t/4439 -> concatenate34/87
  t/4440 -> concatenate34/88
  t/4441 -> concatenate34/89
  t/4442 -> concatenate34/90
  t/4443 -> concatenate34/91
  t/4444 -> concatenate34/92
  t/4445 -> concatenate34/93
  t/4446 -> concatenate34/94
  t/4447 -> concatenate34/95
  t/4448 -> concatenate34/96
  t/4449 -> concatenate34/97
  t/4450 -> concatenate34/98
  t/4451 -> concatenate34/99
  t/4452 -> concatenate34/100
  t/4453 -> concatenate34/101
  t/4454 -> concatenate34/102
  t/4455 -> concatenate34/103
  t/4456 -> concatenate34/104
  t/4457 -> concatenate34/105
  t/4458 -> concatenate34/106
  t/4459 -> concatenate34/107
  t/4460 -> concatenate34/108
  t/4461 -> concatenate34/109
  t/4462 -> concatenate34/110
  t/4463 -> concatenate34/111
  t/4464 -> concatenate34/112
  t/4465 -> concatenate34/113
  t/4466 -> concatenate34/114
  t/4467 -> concatenate34/115
  t/4468 -> concatenate34/116
  t/4469 -> concatenate34/117
  t/4470 -> concatenate34/118
  t/4471 -> concatenate34/119
  t/4472 -> concatenate34/120
  t/4473 -> concatenate34/121
  t/4474 -> concatenate34/122
  t/4475 -> concatenate34/123
  t/4476 -> concatenate34/124
  t/4477 -> concatenate34/125
  t/4478 -> concatenate34/126
  t/4479 -> concatenate34/127
  t/4480 -> concatenate34/128
  t/4481 -> concatenate35/1
  t/4482 -> concatenate35/2
  t/4483 -> concatenate35/3
  t/4484 -> concatenate35/4
  t/4485 -> concatenate35/5
  t/4486 -> concatenate35/6
  t/4487 -> concatenate35/7
  t/4488 -> concatenate35/8
  t/4489 -> concatenate35/9
  t/4490 -> concatenate35/10
  t/4491 -> concatenate35/11
  t/4492 -> concatenate35/12
  t/4493 -> concatenate35/13
  t/4494 -> concatenate35/14
  t/4495 -> concatenate35/15
  t/4496 -> concatenate35/16
  t/4497 -> concatenate35/17
  t/4498 -> concatenate35/18
  t/4499 -> concatenate35/19
  t/4500 -> concatenate35/20
  t/4501 -> concatenate35/21
  t/4502 -> concatenate35/22
  t/4503 -> concatenate35/23
  t/4504 -> concatenate35/24
  t/4505 -> concatenate35/25
  t/4506 -> concatenate35/26
  t/4507 -> concatenate35/27
  t/4508 -> concatenate35/28
  t/4509 -> concatenate35/29
  t/4510 -> concatenate35/30
  t/4511 -> concatenate35/31
  t/4512 -> concatenate35/32
  t/4513 -> concatenate35/33
  t/4514 -> concatenate35/34
  t/4515 -> concatenate35/35
  t/4516 -> concatenate35/36
  t/4517 -> concatenate35/37
  t/4518 -> concatenate35/38
  t/4519 -> concatenate35/39
  t/4520 -> concatenate35/40
  t/4521 -> concatenate35/41
  t/4522 -> concatenate35/42
  t/4523 -> concatenate35/43
  t/4524 -> concatenate35/44
  t/4525 -> concatenate35/45
  t/4526 -> concatenate35/46
  t/4527 -> concatenate35/47
  t/4528 -> concatenate35/48
  t/4529 -> concatenate35/49
  t/4530 -> concatenate35/50
  t/4531 -> concatenate35/51
  t/4532 -> concatenate35/52
  t/4533 -> concatenate35/53
  t/4534 -> concatenate35/54
  t/4535 -> concatenate35/55
  t/4536 -> concatenate35/56
  t/4537 -> concatenate35/57
  t/4538 -> concatenate35/58
  t/4539 -> concatenate35/59
  t/4540 -> concatenate35/60
  t/4541 -> concatenate35/61
  t/4542 -> concatenate35/62
  t/4543 -> concatenate35/63
  t/4544 -> concatenate35/64
  t/4545 -> concatenate35/65
  t/4546 -> concatenate35/66
  t/4547 -> concatenate35/67
  t/4548 -> concatenate35/68
  t/4549 -> concatenate35/69
  t/4550 -> concatenate35/70
  t/4551 -> concatenate35/71
  t/4552 -> concatenate35/72
  t/4553 -> concatenate35/73
  t/4554 -> concatenate35/74
  t/4555 -> concatenate35/75
  t/4556 -> concatenate35/76
  t/4557 -> concatenate35/77
  t/4558 -> concatenate35/78
  t/4559 -> concatenate35/79
  t/4560 -> concatenate35/80
  t/4561 -> concatenate35/81
  t/4562 -> concatenate35/82
  t/4563 -> concatenate35/83
  t/4564 -> concatenate35/84
  t/4565 -> concatenate35/85
  t/4566 -> concatenate35/86
  t/4567 -> concatenate35/87
  t/4568 -> concatenate35/88
  t/4569 -> concatenate35/89
  t/4570 -> concatenate35/90
  t/4571 -> concatenate35/91
  t/4572 -> concatenate35/92
  t/4573 -> concatenate35/93
  t/4574 -> concatenate35/94
  t/4575 -> concatenate35/95
  t/4576 -> concatenate35/96
  t/4577 -> concatenate35/97
  t/4578 -> concatenate35/98
  t/4579 -> concatenate35/99
  t/4580 -> concatenate35/100
  t/4581 -> concatenate35/101
  t/4582 -> concatenate35/102
  t/4583 -> concatenate35/103
  t/4584 -> concatenate35/104
  t/4585 -> concatenate35/105
  t/4586 -> concatenate35/106
  t/4587 -> concatenate35/107
  t/4588 -> concatenate35/108
  t/4589 -> concatenate35/109
  t/4590 -> concatenate35/110
  t/4591 -> concatenate35/111
  t/4592 -> concatenate35/112
  t/4593 -> concatenate35/113
  t/4594 -> concatenate35/114
  t/4595 -> concatenate35/115
  t/4596 -> concatenate35/116
  t/4597 -> concatenate35/117
  t/4598 -> concatenate35/118
  t/4599 -> concatenate35/119
  t/4600 -> concatenate35/120
  t/4601 -> concatenate35/121
  t/4602 -> concatenate35/122
  t/4603 -> concatenate35/123
  t/4604 -> concatenate35/124
  t/4605 -> concatenate35/125
  t/4606 -> concatenate35/126
  t/4607 -> concatenate35/127
  t/4608 -> concatenate35/128
  t/4609 -> concatenate36/1
  t/4610 -> concatenate36/2
  t/4611 -> concatenate36/3
  t/4612 -> concatenate36/4
  t/4613 -> concatenate36/5
  t/4614 -> concatenate36/6
  t/4615 -> concatenate36/7
  t/4616 -> concatenate36/8
  t/4617 -> concatenate36/9
  t/4618 -> concatenate36/10
  t/4619 -> concatenate36/11
  t/4620 -> concatenate36/12
  t/4621 -> concatenate36/13
  t/4622 -> concatenate36/14
  t/4623 -> concatenate36/15
  t/4624 -> concatenate36/16
  t/4625 -> concatenate36/17
  t/4626 -> concatenate36/18
  t/4627 -> concatenate36/19
  t/4628 -> concatenate36/20
  t/4629 -> concatenate36/21
  t/4630 -> concatenate36/22
  t/4631 -> concatenate36/23
  t/4632 -> concatenate36/24
  t/4633 -> concatenate36/25
  t/4634 -> concatenate36/26
  t/4635 -> concatenate36/27
  t/4636 -> concatenate36/28
  t/4637 -> concatenate36/29
  t/4638 -> concatenate36/30
  t/4639 -> concatenate36/31
  t/4640 -> concatenate36/32
  t/4641 -> concatenate36/33
  t/4642 -> concatenate36/34
  t/4643 -> concatenate36/35
  t/4644 -> concatenate36/36
  t/4645 -> concatenate36/37
  t/4646 -> concatenate36/38
  t/4647 -> concatenate36/39
  t/4648 -> concatenate36/40
  t/4649 -> concatenate36/41
  t/4650 -> concatenate36/42
  t/4651 -> concatenate36/43
  t/4652 -> concatenate36/44
  t/4653 -> concatenate36/45
  t/4654 -> concatenate36/46
  t/4655 -> concatenate36/47
  t/4656 -> concatenate36/48
  t/4657 -> concatenate36/49
  t/4658 -> concatenate36/50
  t/4659 -> concatenate36/51
  t/4660 -> concatenate36/52
  t/4661 -> concatenate36/53
  t/4662 -> concatenate36/54
  t/4663 -> concatenate36/55
  t/4664 -> concatenate36/56
  t/4665 -> concatenate36/57
  t/4666 -> concatenate36/58
  t/4667 -> concatenate36/59
  t/4668 -> concatenate36/60
  t/4669 -> concatenate36/61
  t/4670 -> concatenate36/62
  t/4671 -> concatenate36/63
  t/4672 -> concatenate36/64
  t/4673 -> concatenate36/65
  t/4674 -> concatenate36/66
  t/4675 -> concatenate36/67
  t/4676 -> concatenate36/68
  t/4677 -> concatenate36/69
  t/4678 -> concatenate36/70
  t/4679 -> concatenate36/71
  t/4680 -> concatenate36/72
  t/4681 -> concatenate36/73
  t/4682 -> concatenate36/74
  t/4683 -> concatenate36/75
  t/4684 -> concatenate36/76
  t/4685 -> concatenate36/77
  t/4686 -> concatenate36/78
  t/4687 -> concatenate36/79
  t/4688 -> concatenate36/80
  t/4689 -> concatenate36/81
  t/4690 -> concatenate36/82
  t/4691 -> concatenate36/83
  t/4692 -> concatenate36/84
  t/4693 -> concatenate36/85
  t/4694 -> concatenate36/86
  t/4695 -> concatenate36/87
  t/4696 -> concatenate36/88
  t/4697 -> concatenate36/89
  t/4698 -> concatenate36/90
  t/4699 -> concatenate36/91
  t/4700 -> concatenate36/92
  t/4701 -> concatenate36/93
  t/4702 -> concatenate36/94
  t/4703 -> concatenate36/95
  t/4704 -> concatenate36/96
  t/4705 -> concatenate36/97
  t/4706 -> concatenate36/98
  t/4707 -> concatenate36/99
  t/4708 -> concatenate36/100
  t/4709 -> concatenate36/101
  t/4710 -> concatenate36/102
  t/4711 -> concatenate36/103
  t/4712 -> concatenate36/104
  t/4713 -> concatenate36/105
  t/4714 -> concatenate36/106
  t/4715 -> concatenate36/107
  t/4716 -> concatenate36/108
  t/4717 -> concatenate36/109
  t/4718 -> concatenate36/110
  t/4719 -> concatenate36/111
  t/4720 -> concatenate36/112
  t/4721 -> concatenate36/113
  t/4722 -> concatenate36/114
  t/4723 -> concatenate36/115
  t/4724 -> concatenate36/116
  t/4725 -> concatenate36/117
  t/4726 -> concatenate36/118
  t/4727 -> concatenate36/119
  t/4728 -> concatenate36/120
  t/4729 -> concatenate36/121
  t/4730 -> concatenate36/122
  t/4731 -> concatenate36/123
  t/4732 -> concatenate36/124
  t/4733 -> concatenate36/125
  t/4734 -> concatenate36/126
  t/4735 -> concatenate36/127
  t/4736 -> concatenate36/128
  t/4737 -> concatenate37/1
  t/4738 -> concatenate37/2
  t/4739 -> concatenate37/3
  t/4740 -> concatenate37/4
  t/4741 -> concatenate37/5
  t/4742 -> concatenate37/6
  t/4743 -> concatenate37/7
  t/4744 -> concatenate37/8
  t/4745 -> concatenate37/9
  t/4746 -> concatenate37/10
  t/4747 -> concatenate37/11
  t/4748 -> concatenate37/12
  t/4749 -> concatenate37/13
  t/4750 -> concatenate37/14
  t/4751 -> concatenate37/15
  t/4752 -> concatenate37/16
  t/4753 -> concatenate37/17
  t/4754 -> concatenate37/18
  t/4755 -> concatenate37/19
  t/4756 -> concatenate37/20
  t/4757 -> concatenate37/21
  t/4758 -> concatenate37/22
  t/4759 -> concatenate37/23
  t/4760 -> concatenate37/24
  t/4761 -> concatenate37/25
  t/4762 -> concatenate37/26
  t/4763 -> concatenate37/27
  t/4764 -> concatenate37/28
  t/4765 -> concatenate37/29
  t/4766 -> concatenate37/30
  t/4767 -> concatenate37/31
  t/4768 -> concatenate37/32
  t/4769 -> concatenate37/33
  t/4770 -> concatenate37/34
  t/4771 -> concatenate37/35
  t/4772 -> concatenate37/36
  t/4773 -> concatenate37/37
  t/4774 -> concatenate37/38
  t/4775 -> concatenate37/39
  t/4776 -> concatenate37/40
  t/4777 -> concatenate37/41
  t/4778 -> concatenate37/42
  t/4779 -> concatenate37/43
  t/4780 -> concatenate37/44
  t/4781 -> concatenate37/45
  t/4782 -> concatenate37/46
  t/4783 -> concatenate37/47
  t/4784 -> concatenate37/48
  t/4785 -> concatenate37/49
  t/4786 -> concatenate37/50
  t/4787 -> concatenate37/51
  t/4788 -> concatenate37/52
  t/4789 -> concatenate37/53
  t/4790 -> concatenate37/54
  t/4791 -> concatenate37/55
  t/4792 -> concatenate37/56
  t/4793 -> concatenate37/57
  t/4794 -> concatenate37/58
  t/4795 -> concatenate37/59
  t/4796 -> concatenate37/60
  t/4797 -> concatenate37/61
  t/4798 -> concatenate37/62
  t/4799 -> concatenate37/63
  t/4800 -> concatenate37/64
  t/4801 -> concatenate37/65
  t/4802 -> concatenate37/66
  t/4803 -> concatenate37/67
  t/4804 -> concatenate37/68
  t/4805 -> concatenate37/69
  t/4806 -> concatenate37/70
  t/4807 -> concatenate37/71
  t/4808 -> concatenate37/72
  t/4809 -> concatenate37/73
  t/4810 -> concatenate37/74
  t/4811 -> concatenate37/75
  t/4812 -> concatenate37/76
  t/4813 -> concatenate37/77
  t/4814 -> concatenate37/78
  t/4815 -> concatenate37/79
  t/4816 -> concatenate37/80
  t/4817 -> concatenate37/81
  t/4818 -> concatenate37/82
  t/4819 -> concatenate37/83
  t/4820 -> concatenate37/84
  t/4821 -> concatenate37/85
  t/4822 -> concatenate37/86
  t/4823 -> concatenate37/87
  t/4824 -> concatenate37/88
  t/4825 -> concatenate37/89
  t/4826 -> concatenate37/90
  t/4827 -> concatenate37/91
  t/4828 -> concatenate37/92
  t/4829 -> concatenate37/93
  t/4830 -> concatenate37/94
  t/4831 -> concatenate37/95
  t/4832 -> concatenate37/96
  t/4833 -> concatenate37/97
  t/4834 -> concatenate37/98
  t/4835 -> concatenate37/99
  t/4836 -> concatenate37/100
  t/4837 -> concatenate37/101
  t/4838 -> concatenate37/102
  t/4839 -> concatenate37/103
  t/4840 -> concatenate37/104
  t/4841 -> concatenate37/105
  t/4842 -> concatenate37/106
  t/4843 -> concatenate37/107
  t/4844 -> concatenate37/108
